simulink model "model"  (R2014a)
(part 5 of 6)

  bus544 : powerlib/Measurements/Load Flow Bus  LConnTagsString=a  ID=bus544  Vbase=132000  Vref=1  Vangle=0  VLF=1  angleLF=0
      settings: AttributesFormatString=|
      | %<ID>
      | %<Vbase>V
      | %<VLF>pu
      | %<angleLF>deg.
      | %<Name>
  bus545 : powerlib/Measurements/Load Flow Bus  LConnTagsString=a  ID=bus545  Vbase=132000  Vref=1  Vangle=0  VLF=1  angleLF=0
      settings: AttributesFormatString=|
      | %<ID>
      | %<Vbase>V
      | %<VLF>pu
      | %<angleLF>deg.
      | %<Name>
  bus546 : powerlib/Measurements/Load Flow Bus  LConnTagsString=a  ID=bus546  Vbase=132000  Vref=1  Vangle=0  VLF=1  angleLF=0
      settings: AttributesFormatString=|
      | %<ID>
      | %<Vbase>V
      | %<VLF>pu
      | %<angleLF>deg.
      | %<Name>
  bus547 : powerlib/Measurements/Load Flow Bus  LConnTagsString=a  ID=bus547  Vbase=132000  Vref=1  Vangle=0  VLF=1  angleLF=0
      settings: AttributesFormatString=|
      | %<ID>
      | %<Vbase>V
      | %<VLF>pu
      | %<angleLF>deg.
      | %<Name>
  bus548 : powerlib/Measurements/Load Flow Bus  LConnTagsString=a  ID=bus548  Vbase=132000  Vref=1  Vangle=0  VLF=1  angleLF=0
      settings: AttributesFormatString=|
      | %<ID>
      | %<Vbase>V
      | %<VLF>pu
      | %<angleLF>deg.
      | %<Name>
  bus549 : powerlib/Measurements/Load Flow Bus  LConnTagsString=a  ID=bus549  Vbase=132000  Vref=1  Vangle=0  VLF=1  angleLF=0
      settings: AttributesFormatString=|
      | %<ID>
      | %<Vbase>V
      | %<VLF>pu
      | %<angleLF>deg.
      | %<Name>
  bus55 : powerlib/Measurements/Load Flow Bus  LConnTagsString=a  ID=bus55  Vbase=132000  Vref=1  Vangle=0  VLF=1  angleLF=0
      settings: AttributesFormatString=|
      | %<ID>
      | %<Vbase>V
      | %<VLF>pu
      | %<angleLF>deg.
      | %<Name>
  bus550 : powerlib/Measurements/Load Flow Bus  LConnTagsString=a  ID=bus550  Vbase=132000  Vref=1  Vangle=0  VLF=1  angleLF=0
      settings: AttributesFormatString=|
      | %<ID>
      | %<Vbase>V
      | %<VLF>pu
      | %<angleLF>deg.
      | %<Name>
  bus551 : powerlib/Measurements/Load Flow Bus  LConnTagsString=a  ID=bus551  Vbase=132000  Vref=1  Vangle=0  VLF=1  angleLF=0
      settings: AttributesFormatString=|
      | %<ID>
      | %<Vbase>V
      | %<VLF>pu
      | %<angleLF>deg.
      | %<Name>
  bus552 : powerlib/Measurements/Load Flow Bus  LConnTagsString=a  ID=bus552  Vbase=132000  Vref=1  Vangle=0  VLF=1  angleLF=0
      settings: AttributesFormatString=|
      | %<ID>
      | %<Vbase>V
      | %<VLF>pu
      | %<angleLF>deg.
      | %<Name>
  bus553 : powerlib/Measurements/Load Flow Bus  LConnTagsString=a  ID=bus553  Vbase=132000  Vref=1  Vangle=0  VLF=1  angleLF=0
      settings: AttributesFormatString=|
      | %<ID>
      | %<Vbase>V
      | %<VLF>pu
      | %<angleLF>deg.
      | %<Name>
  bus554 : powerlib/Measurements/Load Flow Bus  LConnTagsString=a  ID=bus554  Vbase=132000  Vref=1  Vangle=0  VLF=1  angleLF=0
      settings: AttributesFormatString=|
      | %<ID>
      | %<Vbase>V
      | %<VLF>pu
      | %<angleLF>deg.
      | %<Name>
  bus555 : powerlib/Measurements/Load Flow Bus  LConnTagsString=a  ID=bus555  Vbase=132000  Vref=1  Vangle=0  VLF=1  angleLF=0
      settings: AttributesFormatString=|
      | %<ID>
      | %<Vbase>V
      | %<VLF>pu
      | %<angleLF>deg.
      | %<Name>
  bus556 : powerlib/Measurements/Load Flow Bus  LConnTagsString=a  ID=bus556  Vbase=220000  Vref=1  Vangle=0  VLF=1  angleLF=0
      settings: AttributesFormatString=|
      | %<ID>
      | %<Vbase>V
      | %<VLF>pu
      | %<angleLF>deg.
      | %<Name>
  bus557 : powerlib/Measurements/Load Flow Bus  LConnTagsString=a  ID=bus557  Vbase=220000  Vref=1  Vangle=0  VLF=1  angleLF=0
      settings: AttributesFormatString=|
      | %<ID>
      | %<Vbase>V
      | %<VLF>pu
      | %<angleLF>deg.
      | %<Name>
  bus558 : powerlib/Measurements/Load Flow Bus  LConnTagsString=a  ID=bus558  Vbase=220000  Vref=1  Vangle=0  VLF=1  angleLF=0
      settings: AttributesFormatString=|
      | %<ID>
      | %<Vbase>V
      | %<VLF>pu
      | %<angleLF>deg.
      | %<Name>
  bus559 : powerlib/Measurements/Load Flow Bus  LConnTagsString=a  ID=bus559  Vbase=220000  Vref=1  Vangle=0  VLF=1  angleLF=0
      settings: AttributesFormatString=|
      | %<ID>
      | %<Vbase>V
      | %<VLF>pu
      | %<angleLF>deg.
      | %<Name>
  bus56 : powerlib/Measurements/Load Flow Bus  LConnTagsString=a  ID=bus56  Vbase=132000  Vref=1  Vangle=0  VLF=1  angleLF=0
      settings: AttributesFormatString=|
      | %<ID>
      | %<Vbase>V
      | %<VLF>pu
      | %<angleLF>deg.
      | %<Name>
  bus560 : powerlib/Measurements/Load Flow Bus  LConnTagsString=a  ID=bus560  Vbase=220000  Vref=1  Vangle=0  VLF=1  angleLF=0
      settings: AttributesFormatString=|
      | %<ID>
      | %<Vbase>V
      | %<VLF>pu
      | %<angleLF>deg.
      | %<Name>
  bus561 : powerlib/Measurements/Load Flow Bus  LConnTagsString=a  ID=bus561  Vbase=220000  Vref=1  Vangle=0  VLF=1  angleLF=0
      settings: AttributesFormatString=|
      | %<ID>
      | %<Vbase>V
      | %<VLF>pu
      | %<angleLF>deg.
      | %<Name>
  bus562 : powerlib/Measurements/Load Flow Bus  LConnTagsString=a  ID=bus562  Vbase=220000  Vref=1  Vangle=0  VLF=1  angleLF=0
      settings: AttributesFormatString=|
      | %<ID>
      | %<Vbase>V
      | %<VLF>pu
      | %<angleLF>deg.
      | %<Name>
  bus563 : powerlib/Measurements/Load Flow Bus  LConnTagsString=a  ID=bus563  Vbase=220000  Vref=1  Vangle=0  VLF=1  angleLF=0
      settings: AttributesFormatString=|
      | %<ID>
      | %<Vbase>V
      | %<VLF>pu
      | %<angleLF>deg.
      | %<Name>
  bus564 : powerlib/Measurements/Load Flow Bus  LConnTagsString=a  ID=bus564  Vbase=220000  Vref=1  Vangle=0  VLF=1  angleLF=0
      settings: AttributesFormatString=|
      | %<ID>
      | %<Vbase>V
      | %<VLF>pu
      | %<angleLF>deg.
      | %<Name>
  bus565 : powerlib/Measurements/Load Flow Bus  LConnTagsString=a  ID=bus565  Vbase=220000  Vref=1  Vangle=0  VLF=1  angleLF=0
      settings: AttributesFormatString=|
      | %<ID>
      | %<Vbase>V
      | %<VLF>pu
      | %<angleLF>deg.
      | %<Name>
  bus566 : powerlib/Measurements/Load Flow Bus  LConnTagsString=a  ID=bus566  Vbase=220000  Vref=1  Vangle=0  VLF=1  angleLF=0
      settings: AttributesFormatString=|
      | %<ID>
      | %<Vbase>V
      | %<VLF>pu
      | %<angleLF>deg.
      | %<Name>
  bus567 : powerlib/Measurements/Load Flow Bus  LConnTagsString=a  ID=bus567  Vbase=220000  Vref=1  Vangle=0  VLF=1  angleLF=0
      settings: AttributesFormatString=|
      | %<ID>
      | %<Vbase>V
      | %<VLF>pu
      | %<angleLF>deg.
      | %<Name>
  bus568 : powerlib/Measurements/Load Flow Bus  LConnTagsString=a  ID=bus568  Vbase=220000  Vref=1  Vangle=0  VLF=1  angleLF=0
      settings: AttributesFormatString=|
      | %<ID>
      | %<Vbase>V
      | %<VLF>pu
      | %<angleLF>deg.
      | %<Name>
  bus569 : powerlib/Measurements/Load Flow Bus  LConnTagsString=a  ID=bus569  Vbase=220000  Vref=1  Vangle=0  VLF=1  angleLF=0
      settings: AttributesFormatString=|
      | %<ID>
      | %<Vbase>V
      | %<VLF>pu
      | %<angleLF>deg.
      | %<Name>
  bus57 : powerlib/Measurements/Load Flow Bus  LConnTagsString=a  ID=bus57  Vbase=132000  Vref=1  Vangle=0  VLF=1  angleLF=0
      settings: AttributesFormatString=|
      | %<ID>
      | %<Vbase>V
      | %<VLF>pu
      | %<angleLF>deg.
      | %<Name>
  bus570 : powerlib/Measurements/Load Flow Bus  LConnTagsString=a  ID=bus570  Vbase=220000  Vref=1  Vangle=0  VLF=1  angleLF=0
      settings: AttributesFormatString=|
      | %<ID>
      | %<Vbase>V
      | %<VLF>pu
      | %<angleLF>deg.
      | %<Name>
  bus571 : powerlib/Measurements/Load Flow Bus  LConnTagsString=a  ID=bus571  Vbase=220000  Vref=1  Vangle=0  VLF=1  angleLF=0
      settings: AttributesFormatString=|
      | %<ID>
      | %<Vbase>V
      | %<VLF>pu
      | %<angleLF>deg.
      | %<Name>
  bus572 : powerlib/Measurements/Load Flow Bus  LConnTagsString=a  ID=bus572  Vbase=220000  Vref=1  Vangle=0  VLF=1  angleLF=0
      settings: AttributesFormatString=|
      | %<ID>
      | %<Vbase>V
      | %<VLF>pu
      | %<angleLF>deg.
      | %<Name>
  bus573 : powerlib/Measurements/Load Flow Bus  LConnTagsString=a  ID=bus573  Vbase=220000  Vref=1  Vangle=0  VLF=1  angleLF=0
      settings: AttributesFormatString=|
      | %<ID>
      | %<Vbase>V
      | %<VLF>pu
      | %<angleLF>deg.
      | %<Name>
  bus574 : powerlib/Measurements/Load Flow Bus  LConnTagsString=a  ID=bus574  Vbase=220000  Vref=1  Vangle=0  VLF=1  angleLF=0
      settings: AttributesFormatString=|
      | %<ID>
      | %<Vbase>V
      | %<VLF>pu
      | %<angleLF>deg.
      | %<Name>
  bus575 : powerlib/Measurements/Load Flow Bus  LConnTagsString=a  ID=bus575  Vbase=220000  Vref=1  Vangle=0  VLF=1  angleLF=0
      settings: AttributesFormatString=|
      | %<ID>
      | %<Vbase>V
      | %<VLF>pu
      | %<angleLF>deg.
      | %<Name>
  bus576 : powerlib/Measurements/Load Flow Bus  LConnTagsString=a  ID=bus576  Vbase=220000  Vref=1  Vangle=0  VLF=1  angleLF=0
      settings: AttributesFormatString=|
      | %<ID>
      | %<Vbase>V
      | %<VLF>pu
      | %<angleLF>deg.
      | %<Name>
  bus577 : powerlib/Measurements/Load Flow Bus  LConnTagsString=a  ID=bus577  Vbase=220000  Vref=1  Vangle=0  VLF=1  angleLF=0
      settings: AttributesFormatString=|
      | %<ID>
      | %<Vbase>V
      | %<VLF>pu
      | %<angleLF>deg.
      | %<Name>
  bus578 : powerlib/Measurements/Load Flow Bus  LConnTagsString=a  ID=bus578  Vbase=220000  Vref=1  Vangle=0  VLF=1  angleLF=0
      settings: AttributesFormatString=|
      | %<ID>
      | %<Vbase>V
      | %<VLF>pu
      | %<angleLF>deg.
      | %<Name>
  bus579 : powerlib/Measurements/Load Flow Bus  LConnTagsString=a  ID=bus579  Vbase=220000  Vref=1  Vangle=0  VLF=1  angleLF=0
      settings: AttributesFormatString=|
      | %<ID>
      | %<Vbase>V
      | %<VLF>pu
      | %<angleLF>deg.
      | %<Name>
  bus58 : powerlib/Measurements/Load Flow Bus  LConnTagsString=a  ID=bus58  Vbase=132000  Vref=1  Vangle=0  VLF=1  angleLF=0
      settings: AttributesFormatString=|
      | %<ID>
      | %<Vbase>V
      | %<VLF>pu
      | %<angleLF>deg.
      | %<Name>
  bus580 : powerlib/Measurements/Load Flow Bus  LConnTagsString=a  ID=bus580  Vbase=220000  Vref=1  Vangle=0  VLF=1  angleLF=0
      settings: AttributesFormatString=|
      | %<ID>
      | %<Vbase>V
      | %<VLF>pu
      | %<angleLF>deg.
      | %<Name>
  bus581 : powerlib/Measurements/Load Flow Bus  LConnTagsString=a  ID=bus581  Vbase=220000  Vref=1  Vangle=0  VLF=1  angleLF=0
      settings: AttributesFormatString=|
      | %<ID>
      | %<Vbase>V
      | %<VLF>pu
      | %<angleLF>deg.
      | %<Name>
  bus582 : powerlib/Measurements/Load Flow Bus  LConnTagsString=a  ID=bus582  Vbase=220000  Vref=1  Vangle=0  VLF=1  angleLF=0
      settings: AttributesFormatString=|
      | %<ID>
      | %<Vbase>V
      | %<VLF>pu
      | %<angleLF>deg.
      | %<Name>
  bus583 : powerlib/Measurements/Load Flow Bus  LConnTagsString=a  ID=bus583  Vbase=220000  Vref=1  Vangle=0  VLF=1  angleLF=0
      settings: AttributesFormatString=|
      | %<ID>
      | %<Vbase>V
      | %<VLF>pu
      | %<angleLF>deg.
      | %<Name>
  bus584 : powerlib/Measurements/Load Flow Bus  LConnTagsString=a  ID=bus584  Vbase=220000  Vref=1  Vangle=0  VLF=1  angleLF=0
      settings: AttributesFormatString=|
      | %<ID>
      | %<Vbase>V
      | %<VLF>pu
      | %<angleLF>deg.
      | %<Name>
  bus585 : powerlib/Measurements/Load Flow Bus  LConnTagsString=a  ID=bus585  Vbase=220000  Vref=1  Vangle=0  VLF=1  angleLF=0
      settings: AttributesFormatString=|
      | %<ID>
      | %<Vbase>V
      | %<VLF>pu
      | %<angleLF>deg.
      | %<Name>
  bus586 : powerlib/Measurements/Load Flow Bus  LConnTagsString=a  ID=bus586  Vbase=230000  Vref=1  Vangle=0  VLF=1  angleLF=0
      settings: AttributesFormatString=|
      | %<ID>
      | %<Vbase>V
      | %<VLF>pu
      | %<angleLF>deg.
      | %<Name>
  bus587 : powerlib/Measurements/Load Flow Bus  LConnTagsString=a  ID=bus587  Vbase=230000  Vref=1  Vangle=0  VLF=1  angleLF=0
      settings: AttributesFormatString=|
      | %<ID>
      | %<Vbase>V
      | %<VLF>pu
      | %<angleLF>deg.
      | %<Name>
  bus588 : powerlib/Measurements/Load Flow Bus  LConnTagsString=a  ID=bus588  Vbase=230000  Vref=1  Vangle=0  VLF=1  angleLF=0
      settings: AttributesFormatString=|
      | %<ID>
      | %<Vbase>V
      | %<VLF>pu
      | %<angleLF>deg.
      | %<Name>
  bus589 : powerlib/Measurements/Load Flow Bus  LConnTagsString=a  ID=bus589  Vbase=230000  Vref=1  Vangle=0  VLF=1  angleLF=0
      settings: AttributesFormatString=|
      | %<ID>
      | %<Vbase>V
      | %<VLF>pu
      | %<angleLF>deg.
      | %<Name>
  bus59 : powerlib/Measurements/Load Flow Bus  LConnTagsString=a  ID=bus59  Vbase=132000  Vref=1  Vangle=0  VLF=1  angleLF=0
      settings: AttributesFormatString=|
      | %<ID>
      | %<Vbase>V
      | %<VLF>pu
      | %<angleLF>deg.
      | %<Name>
  bus590 : powerlib/Measurements/Load Flow Bus  LConnTagsString=a  ID=bus590  Vbase=230000  Vref=1  Vangle=0  VLF=1  angleLF=0
      settings: AttributesFormatString=|
      | %<ID>
      | %<Vbase>V
      | %<VLF>pu
      | %<angleLF>deg.
      | %<Name>
  bus591 : powerlib/Measurements/Load Flow Bus  LConnTagsString=a  ID=bus591  Vbase=230000  Vref=1  Vangle=0  VLF=1  angleLF=0
      settings: AttributesFormatString=|
      | %<ID>
      | %<Vbase>V
      | %<VLF>pu
      | %<angleLF>deg.
      | %<Name>
  bus592 : powerlib/Measurements/Load Flow Bus  LConnTagsString=a  ID=bus592  Vbase=230000  Vref=1  Vangle=0  VLF=1  angleLF=0
      settings: AttributesFormatString=|
      | %<ID>
      | %<Vbase>V
      | %<VLF>pu
      | %<angleLF>deg.
      | %<Name>
  bus593 : powerlib/Measurements/Load Flow Bus  LConnTagsString=a  ID=bus593  Vbase=230000  Vref=1  Vangle=0  VLF=1  angleLF=0
      settings: AttributesFormatString=|
      | %<ID>
      | %<Vbase>V
      | %<VLF>pu
      | %<angleLF>deg.
      | %<Name>
  bus594 : powerlib/Measurements/Load Flow Bus  LConnTagsString=a  ID=bus594  Vbase=230000  Vref=1  Vangle=0  VLF=1  angleLF=0
      settings: AttributesFormatString=|
      | %<ID>
      | %<Vbase>V
      | %<VLF>pu
      | %<angleLF>deg.
      | %<Name>
  bus595 : powerlib/Measurements/Load Flow Bus  LConnTagsString=a  ID=bus595  Vbase=230000  Vref=1  Vangle=0  VLF=1  angleLF=0
      settings: AttributesFormatString=|
      | %<ID>
      | %<Vbase>V
      | %<VLF>pu
      | %<angleLF>deg.
      | %<Name>
  bus596 : powerlib/Measurements/Load Flow Bus  LConnTagsString=a  ID=bus596  Vbase=230000  Vref=1  Vangle=0  VLF=1  angleLF=0
      settings: AttributesFormatString=|
      | %<ID>
      | %<Vbase>V
      | %<VLF>pu
      | %<angleLF>deg.
      | %<Name>
  bus597 : powerlib/Measurements/Load Flow Bus  LConnTagsString=a  ID=bus597  Vbase=230000  Vref=1  Vangle=0  VLF=1  angleLF=0
      settings: AttributesFormatString=|
      | %<ID>
      | %<Vbase>V
      | %<VLF>pu
      | %<angleLF>deg.
      | %<Name>
  bus598 : powerlib/Measurements/Load Flow Bus  LConnTagsString=a  ID=bus598  Vbase=230000  Vref=1  Vangle=0  VLF=1  angleLF=0
      settings: AttributesFormatString=|
      | %<ID>
      | %<Vbase>V
      | %<VLF>pu
      | %<angleLF>deg.
      | %<Name>
  bus599 : powerlib/Measurements/Load Flow Bus  LConnTagsString=a  ID=bus599  Vbase=230000  Vref=1  Vangle=0  VLF=1  angleLF=0
      settings: AttributesFormatString=|
      | %<ID>
      | %<Vbase>V
      | %<VLF>pu
      | %<angleLF>deg.
      | %<Name>
  bus6 : powerlib/Measurements/Load Flow Bus  LConnTagsString=a  ID=bus6  Vbase=132000  Vref=1  Vangle=0  VLF=1  angleLF=0
      settings: AttributesFormatString=|
      | %<ID>
      | %<Vbase>V
      | %<VLF>pu
      | %<angleLF>deg.
      | %<Name>
  bus60 : powerlib/Measurements/Load Flow Bus  LConnTagsString=a  ID=bus60  Vbase=132000  Vref=1  Vangle=0  VLF=1  angleLF=0
      settings: AttributesFormatString=|
      | %<ID>
      | %<Vbase>V
      | %<VLF>pu
      | %<angleLF>deg.
      | %<Name>
  bus600 : powerlib/Measurements/Load Flow Bus  LConnTagsString=a  ID=bus600  Vbase=230000  Vref=1  Vangle=0  VLF=1  angleLF=0
      settings: AttributesFormatString=|
      | %<ID>
      | %<Vbase>V
      | %<VLF>pu
      | %<angleLF>deg.
      | %<Name>
  bus601 : powerlib/Measurements/Load Flow Bus  LConnTagsString=a  ID=bus601  Vbase=230000  Vref=1  Vangle=0  VLF=1  angleLF=0
      settings: AttributesFormatString=|
      | %<ID>
      | %<Vbase>V
      | %<VLF>pu
      | %<angleLF>deg.
      | %<Name>
  bus602 : powerlib/Measurements/Load Flow Bus  LConnTagsString=a  ID=bus602  Vbase=230000  Vref=1  Vangle=0  VLF=1  angleLF=0
      settings: AttributesFormatString=|
      | %<ID>
      | %<Vbase>V
      | %<VLF>pu
      | %<angleLF>deg.
      | %<Name>
  bus603 : powerlib/Measurements/Load Flow Bus  LConnTagsString=a  ID=bus603  Vbase=230000  Vref=1  Vangle=0  VLF=1  angleLF=0
      settings: AttributesFormatString=|
      | %<ID>
      | %<Vbase>V
      | %<VLF>pu
      | %<angleLF>deg.
      | %<Name>
  bus604 : powerlib/Measurements/Load Flow Bus  LConnTagsString=a  ID=bus604  Vbase=230000  Vref=1  Vangle=0  VLF=1  angleLF=0
      settings: AttributesFormatString=|
      | %<ID>
      | %<Vbase>V
      | %<VLF>pu
      | %<angleLF>deg.
      | %<Name>
  bus605 : powerlib/Measurements/Load Flow Bus  LConnTagsString=a  ID=bus605  Vbase=230000  Vref=1  Vangle=0  VLF=1  angleLF=0
      settings: AttributesFormatString=|
      | %<ID>
      | %<Vbase>V
      | %<VLF>pu
      | %<angleLF>deg.
      | %<Name>
  bus606 : powerlib/Measurements/Load Flow Bus  LConnTagsString=a  ID=bus606  Vbase=230000  Vref=1  Vangle=0  VLF=1  angleLF=0
      settings: AttributesFormatString=|
      | %<ID>
      | %<Vbase>V
      | %<VLF>pu
      | %<angleLF>deg.
      | %<Name>
  bus607 : powerlib/Measurements/Load Flow Bus  LConnTagsString=a  ID=bus607  Vbase=275000  Vref=1  Vangle=0  VLF=1  angleLF=0
      settings: AttributesFormatString=|
      | %<ID>
      | %<Vbase>V
      | %<VLF>pu
      | %<angleLF>deg.
      | %<Name>
  bus608 : powerlib/Measurements/Load Flow Bus  LConnTagsString=a  ID=bus608  Vbase=275000  Vref=1  Vangle=0  VLF=1  angleLF=0
      settings: AttributesFormatString=|
      | %<ID>
      | %<Vbase>V
      | %<VLF>pu
      | %<angleLF>deg.
      | %<Name>
  bus609 : powerlib/Measurements/Load Flow Bus  LConnTagsString=a  ID=bus609  Vbase=275000  Vref=1  Vangle=0  VLF=1  angleLF=0
      settings: AttributesFormatString=|
      | %<ID>
      | %<Vbase>V
      | %<VLF>pu
      | %<angleLF>deg.
      | %<Name>
  bus61 : powerlib/Measurements/Load Flow Bus  LConnTagsString=a  ID=bus61  Vbase=132000  Vref=1  Vangle=0  VLF=1  angleLF=0
      settings: AttributesFormatString=|
      | %<ID>
      | %<Vbase>V
      | %<VLF>pu
      | %<angleLF>deg.
      | %<Name>
  bus610 : powerlib/Measurements/Load Flow Bus  LConnTagsString=a  ID=bus610  Vbase=275000  Vref=1  Vangle=0  VLF=1  angleLF=0
      settings: AttributesFormatString=|
      | %<ID>
      | %<Vbase>V
      | %<VLF>pu
      | %<angleLF>deg.
      | %<Name>
  bus611 : powerlib/Measurements/Load Flow Bus  LConnTagsString=a  ID=bus611  Vbase=275000  Vref=1  Vangle=0  VLF=1  angleLF=0
      settings: AttributesFormatString=|
      | %<ID>
      | %<Vbase>V
      | %<VLF>pu
      | %<angleLF>deg.
      | %<Name>
  bus612 : powerlib/Measurements/Load Flow Bus  LConnTagsString=a  ID=bus612  Vbase=275000  Vref=1  Vangle=0  VLF=1  angleLF=0
      settings: AttributesFormatString=|
      | %<ID>
      | %<Vbase>V
      | %<VLF>pu
      | %<angleLF>deg.
      | %<Name>
  bus613 : powerlib/Measurements/Load Flow Bus  LConnTagsString=a  ID=bus613  Vbase=275000  Vref=1  Vangle=0  VLF=1  angleLF=0
      settings: AttributesFormatString=|
      | %<ID>
      | %<Vbase>V
      | %<VLF>pu
      | %<angleLF>deg.
      | %<Name>
  bus614 : powerlib/Measurements/Load Flow Bus  LConnTagsString=a  ID=bus614  Vbase=275000  Vref=1  Vangle=0  VLF=1  angleLF=0
      settings: AttributesFormatString=|
      | %<ID>
      | %<Vbase>V
      | %<VLF>pu
      | %<angleLF>deg.
      | %<Name>
  bus615 : powerlib/Measurements/Load Flow Bus  LConnTagsString=a  ID=bus615  Vbase=275000  Vref=1  Vangle=0  VLF=1  angleLF=0
      settings: AttributesFormatString=|
      | %<ID>
      | %<Vbase>V
      | %<VLF>pu
      | %<angleLF>deg.
      | %<Name>
  bus616 : powerlib/Measurements/Load Flow Bus  LConnTagsString=a  ID=bus616  Vbase=275000  Vref=1  Vangle=0  VLF=1  angleLF=0
      settings: AttributesFormatString=|
      | %<ID>
      | %<Vbase>V
      | %<VLF>pu
      | %<angleLF>deg.
      | %<Name>
  bus617 : powerlib/Measurements/Load Flow Bus  LConnTagsString=a  ID=bus617  Vbase=275000  Vref=1  Vangle=0  VLF=1  angleLF=0
      settings: AttributesFormatString=|
      | %<ID>
      | %<Vbase>V
      | %<VLF>pu
      | %<angleLF>deg.
      | %<Name>
  bus618 : powerlib/Measurements/Load Flow Bus  LConnTagsString=a  ID=bus618  Vbase=275000  Vref=1  Vangle=0  VLF=1  angleLF=0
      settings: AttributesFormatString=|
      | %<ID>
      | %<Vbase>V
      | %<VLF>pu
      | %<angleLF>deg.
      | %<Name>
  bus619 : powerlib/Measurements/Load Flow Bus  LConnTagsString=a  ID=bus619  Vbase=380000  Vref=1  Vangle=0  VLF=1  angleLF=0
      settings: AttributesFormatString=|
      | %<ID>
      | %<Vbase>V
      | %<VLF>pu
      | %<angleLF>deg.
      | %<Name>
  bus62 : powerlib/Measurements/Load Flow Bus  LConnTagsString=a  ID=bus62  Vbase=132000  Vref=1  Vangle=0  VLF=1  angleLF=0
      settings: AttributesFormatString=|
      | %<ID>
      | %<Vbase>V
      | %<VLF>pu
      | %<angleLF>deg.
      | %<Name>
  bus620 : powerlib/Measurements/Load Flow Bus  LConnTagsString=a  ID=bus620  Vbase=380000  Vref=1  Vangle=0  VLF=1  angleLF=0
      settings: AttributesFormatString=|
      | %<ID>
      | %<Vbase>V
      | %<VLF>pu
      | %<angleLF>deg.
      | %<Name>
  bus621 : powerlib/Measurements/Load Flow Bus  LConnTagsString=a  ID=bus621  Vbase=380000  Vref=1  Vangle=0  VLF=1  angleLF=0
      settings: AttributesFormatString=|
      | %<ID>
      | %<Vbase>V
      | %<VLF>pu
      | %<angleLF>deg.
      | %<Name>
  bus622 : powerlib/Measurements/Load Flow Bus  LConnTagsString=a  ID=bus622  Vbase=380000  Vref=1  Vangle=0  VLF=1  angleLF=0
      settings: AttributesFormatString=|
      | %<ID>
      | %<Vbase>V
      | %<VLF>pu
      | %<angleLF>deg.
      | %<Name>
  bus623 : powerlib/Measurements/Load Flow Bus  LConnTagsString=a  ID=bus623  Vbase=380000  Vref=1  Vangle=0  VLF=1  angleLF=0
      settings: AttributesFormatString=|
      | %<ID>
      | %<Vbase>V
      | %<VLF>pu
      | %<angleLF>deg.
      | %<Name>
  bus624 : powerlib/Measurements/Load Flow Bus  LConnTagsString=a  ID=bus624  Vbase=380000  Vref=1  Vangle=0  VLF=1  angleLF=0
      settings: AttributesFormatString=|
      | %<ID>
      | %<Vbase>V
      | %<VLF>pu
      | %<angleLF>deg.
      | %<Name>
  bus625 : powerlib/Measurements/Load Flow Bus  LConnTagsString=a  ID=bus625  Vbase=380000  Vref=1  Vangle=0  VLF=1  angleLF=0
      settings: AttributesFormatString=|
      | %<ID>
      | %<Vbase>V
      | %<VLF>pu
      | %<angleLF>deg.
      | %<Name>
  bus626 : powerlib/Measurements/Load Flow Bus  LConnTagsString=a  ID=bus626  Vbase=380000  Vref=1  Vangle=0  VLF=1  angleLF=0
      settings: AttributesFormatString=|
      | %<ID>
      | %<Vbase>V
      | %<VLF>pu
      | %<angleLF>deg.
      | %<Name>
  bus627 : powerlib/Measurements/Load Flow Bus  LConnTagsString=a  ID=bus627  Vbase=380000  Vref=1  Vangle=0  VLF=1  angleLF=0
      settings: AttributesFormatString=|
      | %<ID>
      | %<Vbase>V
      | %<VLF>pu
      | %<angleLF>deg.
      | %<Name>
  bus628 : powerlib/Measurements/Load Flow Bus  LConnTagsString=a  ID=bus628  Vbase=380000  Vref=1  Vangle=0  VLF=1  angleLF=0
      settings: AttributesFormatString=|
      | %<ID>
      | %<Vbase>V
      | %<VLF>pu
      | %<angleLF>deg.
      | %<Name>
  bus629 : powerlib/Measurements/Load Flow Bus  LConnTagsString=a  ID=bus629  Vbase=380000  Vref=1  Vangle=0  VLF=1  angleLF=0
      settings: AttributesFormatString=|
      | %<ID>
      | %<Vbase>V
      | %<VLF>pu
      | %<angleLF>deg.
      | %<Name>
  bus63 : powerlib/Measurements/Load Flow Bus  LConnTagsString=a  ID=bus63  Vbase=132000  Vref=1  Vangle=0  VLF=1  angleLF=0
      settings: AttributesFormatString=|
      | %<ID>
      | %<Vbase>V
      | %<VLF>pu
      | %<angleLF>deg.
      | %<Name>
  bus630 : powerlib/Measurements/Load Flow Bus  LConnTagsString=a  ID=bus630  Vbase=380000  Vref=1  Vangle=0  VLF=1  angleLF=0
      settings: AttributesFormatString=|
      | %<ID>
      | %<Vbase>V
      | %<VLF>pu
      | %<angleLF>deg.
      | %<Name>
  bus631 : powerlib/Measurements/Load Flow Bus  LConnTagsString=a  ID=bus631  Vbase=380000  Vref=1  Vangle=0  VLF=1  angleLF=0
      settings: AttributesFormatString=|
      | %<ID>
      | %<Vbase>V
      | %<VLF>pu
      | %<angleLF>deg.
      | %<Name>
  bus632 : powerlib/Measurements/Load Flow Bus  LConnTagsString=a  ID=bus632  Vbase=380000  Vref=1  Vangle=0  VLF=1  angleLF=0
      settings: AttributesFormatString=|
      | %<ID>
      | %<Vbase>V
      | %<VLF>pu
      | %<angleLF>deg.
      | %<Name>
  bus633 : powerlib/Measurements/Load Flow Bus  LConnTagsString=a  ID=bus633  Vbase=380000  Vref=1  Vangle=0  VLF=1  angleLF=0
      settings: AttributesFormatString=|
      | %<ID>
      | %<Vbase>V
      | %<VLF>pu
      | %<angleLF>deg.
      | %<Name>
  bus634 : powerlib/Measurements/Load Flow Bus  LConnTagsString=a  ID=bus634  Vbase=380000  Vref=1  Vangle=0  VLF=1  angleLF=0
      settings: AttributesFormatString=|
      | %<ID>
      | %<Vbase>V
      | %<VLF>pu
      | %<angleLF>deg.
      | %<Name>
  bus635 : powerlib/Measurements/Load Flow Bus  LConnTagsString=a  ID=bus635  Vbase=380000  Vref=1  Vangle=0  VLF=1  angleLF=0
      settings: AttributesFormatString=|
      | %<ID>
      | %<Vbase>V
      | %<VLF>pu
      | %<angleLF>deg.
      | %<Name>
  bus636 : powerlib/Measurements/Load Flow Bus  LConnTagsString=a  ID=bus636  Vbase=380000  Vref=1  Vangle=0  VLF=1  angleLF=0
      settings: AttributesFormatString=|
      | %<ID>
      | %<Vbase>V
      | %<VLF>pu
      | %<angleLF>deg.
      | %<Name>
  bus637 : powerlib/Measurements/Load Flow Bus  LConnTagsString=a  ID=bus637  Vbase=380000  Vref=1  Vangle=0  VLF=1  angleLF=0
      settings: AttributesFormatString=|
      | %<ID>
      | %<Vbase>V
      | %<VLF>pu
      | %<angleLF>deg.
      | %<Name>
  bus638 : powerlib/Measurements/Load Flow Bus  LConnTagsString=a  ID=bus638  Vbase=380000  Vref=1  Vangle=0  VLF=1  angleLF=0
      settings: AttributesFormatString=|
      | %<ID>
      | %<Vbase>V
      | %<VLF>pu
      | %<angleLF>deg.
      | %<Name>
  bus639 : powerlib/Measurements/Load Flow Bus  LConnTagsString=a  ID=bus639  Vbase=380000  Vref=1  Vangle=0  VLF=1  angleLF=0
      settings: AttributesFormatString=|
      | %<ID>
      | %<Vbase>V
      | %<VLF>pu
      | %<angleLF>deg.
      | %<Name>
  bus64 : powerlib/Measurements/Load Flow Bus  LConnTagsString=a  ID=bus64  Vbase=132000  Vref=1  Vangle=0  VLF=1  angleLF=0
      settings: AttributesFormatString=|
      | %<ID>
      | %<Vbase>V
      | %<VLF>pu
      | %<angleLF>deg.
      | %<Name>
  bus640 : powerlib/Measurements/Load Flow Bus  LConnTagsString=a  ID=bus640  Vbase=380000  Vref=1  Vangle=0  VLF=1  angleLF=0
      settings: AttributesFormatString=|
      | %<ID>
      | %<Vbase>V
      | %<VLF>pu
      | %<angleLF>deg.
      | %<Name>
  bus641 : powerlib/Measurements/Load Flow Bus  LConnTagsString=a  ID=bus641  Vbase=380000  Vref=1  Vangle=0  VLF=1  angleLF=0
      settings: AttributesFormatString=|
      | %<ID>
      | %<Vbase>V
      | %<VLF>pu
      | %<angleLF>deg.
      | %<Name>
  bus642 : powerlib/Measurements/Load Flow Bus  LConnTagsString=a  ID=bus642  Vbase=380000  Vref=1  Vangle=0  VLF=1  angleLF=0
      settings: AttributesFormatString=|
      | %<ID>
      | %<Vbase>V
      | %<VLF>pu
      | %<angleLF>deg.
      | %<Name>
  bus643 : powerlib/Measurements/Load Flow Bus  LConnTagsString=a  ID=bus643  Vbase=380000  Vref=1  Vangle=0  VLF=1  angleLF=0
      settings: AttributesFormatString=|
      | %<ID>
      | %<Vbase>V
      | %<VLF>pu
      | %<angleLF>deg.
      | %<Name>
  bus644 : powerlib/Measurements/Load Flow Bus  LConnTagsString=a  ID=bus644  Vbase=380000  Vref=1  Vangle=0  VLF=1  angleLF=0
      settings: AttributesFormatString=|
      | %<ID>
      | %<Vbase>V
      | %<VLF>pu
      | %<angleLF>deg.
      | %<Name>
  bus645 : powerlib/Measurements/Load Flow Bus  LConnTagsString=a  ID=bus645  Vbase=380000  Vref=1  Vangle=0  VLF=1  angleLF=0
      settings: AttributesFormatString=|
      | %<ID>
      | %<Vbase>V
      | %<VLF>pu
      | %<angleLF>deg.
      | %<Name>
  bus646 : powerlib/Measurements/Load Flow Bus  LConnTagsString=a  ID=bus646  Vbase=380000  Vref=1  Vangle=0  VLF=1  angleLF=0
      settings: AttributesFormatString=|
      | %<ID>
      | %<Vbase>V
      | %<VLF>pu
      | %<angleLF>deg.
      | %<Name>
  bus647 : powerlib/Measurements/Load Flow Bus  LConnTagsString=a  ID=bus647  Vbase=380000  Vref=1  Vangle=0  VLF=1  angleLF=0
      settings: AttributesFormatString=|
      | %<ID>
      | %<Vbase>V
      | %<VLF>pu
      | %<angleLF>deg.
      | %<Name>
  bus648 : powerlib/Measurements/Load Flow Bus  LConnTagsString=a  ID=bus648  Vbase=380000  Vref=1  Vangle=0  VLF=1  angleLF=0
      settings: AttributesFormatString=|
      | %<ID>
      | %<Vbase>V
      | %<VLF>pu
      | %<angleLF>deg.
      | %<Name>
  bus649 : powerlib/Measurements/Load Flow Bus  LConnTagsString=a  ID=bus649  Vbase=380000  Vref=1  Vangle=0  VLF=1  angleLF=0
      settings: AttributesFormatString=|
      | %<ID>
      | %<Vbase>V
      | %<VLF>pu
      | %<angleLF>deg.
      | %<Name>
  bus65 : powerlib/Measurements/Load Flow Bus  LConnTagsString=a  ID=bus65  Vbase=132000  Vref=1  Vangle=0  VLF=1  angleLF=0
      settings: AttributesFormatString=|
      | %<ID>
      | %<Vbase>V
      | %<VLF>pu
      | %<angleLF>deg.
      | %<Name>
  bus650 : powerlib/Measurements/Load Flow Bus  LConnTagsString=a  ID=bus650  Vbase=380000  Vref=1  Vangle=0  VLF=1  angleLF=0
      settings: AttributesFormatString=|
      | %<ID>
      | %<Vbase>V
      | %<VLF>pu
      | %<angleLF>deg.
      | %<Name>
  bus651 : powerlib/Measurements/Load Flow Bus  LConnTagsString=a  ID=bus651  Vbase=380000  Vref=1  Vangle=0  VLF=1  angleLF=0
      settings: AttributesFormatString=|
      | %<ID>
      | %<Vbase>V
      | %<VLF>pu
      | %<angleLF>deg.
      | %<Name>
  bus652 : powerlib/Measurements/Load Flow Bus  LConnTagsString=a  ID=bus652  Vbase=380000  Vref=1  Vangle=0  VLF=1  angleLF=0
      settings: AttributesFormatString=|
      | %<ID>
      | %<Vbase>V
      | %<VLF>pu
      | %<angleLF>deg.
      | %<Name>
  bus653 : powerlib/Measurements/Load Flow Bus  LConnTagsString=a  ID=bus653  Vbase=400000  Vref=1  Vangle=0  VLF=1  angleLF=0
      settings: AttributesFormatString=|
      | %<ID>
      | %<Vbase>V
      | %<VLF>pu
      | %<angleLF>deg.
      | %<Name>
  bus654 : powerlib/Measurements/Load Flow Bus  LConnTagsString=a  ID=bus654  Vbase=400000  Vref=1  Vangle=0  VLF=1  angleLF=0
      settings: AttributesFormatString=|
      | %<ID>
      | %<Vbase>V
      | %<VLF>pu
      | %<angleLF>deg.
      | %<Name>
  bus655 : powerlib/Measurements/Load Flow Bus  LConnTagsString=a  ID=bus655  Vbase=400000  Vref=1  Vangle=0  VLF=1  angleLF=0
      settings: AttributesFormatString=|
      | %<ID>
      | %<Vbase>V
      | %<VLF>pu
      | %<angleLF>deg.
      | %<Name>
  bus656 : powerlib/Measurements/Load Flow Bus  LConnTagsString=a  ID=bus656  Vbase=400000  Vref=1  Vangle=0  VLF=1  angleLF=0
      settings: AttributesFormatString=|
      | %<ID>
      | %<Vbase>V
      | %<VLF>pu
      | %<angleLF>deg.
      | %<Name>
  bus657 : powerlib/Measurements/Load Flow Bus  LConnTagsString=a  ID=bus657  Vbase=400000  Vref=1  Vangle=0  VLF=1  angleLF=0
      settings: AttributesFormatString=|
      | %<ID>
      | %<Vbase>V
      | %<VLF>pu
      | %<angleLF>deg.
      | %<Name>
  bus658 : powerlib/Measurements/Load Flow Bus  LConnTagsString=a  ID=bus658  Vbase=400000  Vref=1  Vangle=0  VLF=1  angleLF=0
      settings: AttributesFormatString=|
      | %<ID>
      | %<Vbase>V
      | %<VLF>pu
      | %<angleLF>deg.
      | %<Name>
  bus659 : powerlib/Measurements/Load Flow Bus  LConnTagsString=a  ID=bus659  Vbase=400000  Vref=1  Vangle=0  VLF=1  angleLF=0
      settings: AttributesFormatString=|
      | %<ID>
      | %<Vbase>V
      | %<VLF>pu
      | %<angleLF>deg.
      | %<Name>
  bus66 : powerlib/Measurements/Load Flow Bus  LConnTagsString=a  ID=bus66  Vbase=132000  Vref=1  Vangle=0  VLF=1  angleLF=0
      settings: AttributesFormatString=|
      | %<ID>
      | %<Vbase>V
      | %<VLF>pu
      | %<angleLF>deg.
      | %<Name>
  bus660 : powerlib/Measurements/Load Flow Bus  LConnTagsString=a  ID=bus660  Vbase=400000  Vref=1  Vangle=0  VLF=1  angleLF=0
      settings: AttributesFormatString=|
      | %<ID>
      | %<Vbase>V
      | %<VLF>pu
      | %<angleLF>deg.
      | %<Name>
  bus661 : powerlib/Measurements/Load Flow Bus  LConnTagsString=a  ID=bus661  Vbase=400000  Vref=1  Vangle=0  VLF=1  angleLF=0
      settings: AttributesFormatString=|
      | %<ID>
      | %<Vbase>V
      | %<VLF>pu
      | %<angleLF>deg.
      | %<Name>
  bus662 : powerlib/Measurements/Load Flow Bus  LConnTagsString=a  ID=bus662  Vbase=400000  Vref=1  Vangle=0  VLF=1  angleLF=0
      settings: AttributesFormatString=|
      | %<ID>
      | %<Vbase>V
      | %<VLF>pu
      | %<angleLF>deg.
      | %<Name>
  bus663 : powerlib/Measurements/Load Flow Bus  LConnTagsString=a  ID=bus663  Vbase=400000  Vref=1  Vangle=0  VLF=1  angleLF=0
      settings: AttributesFormatString=|
      | %<ID>
      | %<Vbase>V
      | %<VLF>pu
      | %<angleLF>deg.
      | %<Name>
  bus664 : powerlib/Measurements/Load Flow Bus  LConnTagsString=a  ID=bus664  Vbase=400000  Vref=1  Vangle=0  VLF=1  angleLF=0
      settings: AttributesFormatString=|
      | %<ID>
      | %<Vbase>V
      | %<VLF>pu
      | %<angleLF>deg.
      | %<Name>
  bus665 : powerlib/Measurements/Load Flow Bus  LConnTagsString=a  ID=bus665  Vbase=400000  Vref=1  Vangle=0  VLF=1  angleLF=0
      settings: AttributesFormatString=|
      | %<ID>
      | %<Vbase>V
      | %<VLF>pu
      | %<angleLF>deg.
      | %<Name>
  bus666 : powerlib/Measurements/Load Flow Bus  LConnTagsString=a  ID=bus666  Vbase=400000  Vref=1  Vangle=0  VLF=1  angleLF=0
      settings: AttributesFormatString=|
      | %<ID>
      | %<Vbase>V
      | %<VLF>pu
      | %<angleLF>deg.
      | %<Name>
  bus667 : powerlib/Measurements/Load Flow Bus  LConnTagsString=a  ID=bus667  Vbase=400000  Vref=1  Vangle=0  VLF=1  angleLF=0
      settings: AttributesFormatString=|
      | %<ID>
      | %<Vbase>V
      | %<VLF>pu
      | %<angleLF>deg.
      | %<Name>
  bus668 : powerlib/Measurements/Load Flow Bus  LConnTagsString=a  ID=bus668  Vbase=400000  Vref=1  Vangle=0  VLF=1  angleLF=0
      settings: AttributesFormatString=|
      | %<ID>
      | %<Vbase>V
      | %<VLF>pu
      | %<angleLF>deg.
      | %<Name>
  bus669 : powerlib/Measurements/Load Flow Bus  LConnTagsString=a  ID=bus669  Vbase=400000  Vref=1  Vangle=0  VLF=1  angleLF=0
      settings: AttributesFormatString=|
      | %<ID>
      | %<Vbase>V
      | %<VLF>pu
      | %<angleLF>deg.
      | %<Name>
  bus67 : powerlib/Measurements/Load Flow Bus  LConnTagsString=a  ID=bus67  Vbase=132000  Vref=1  Vangle=0  VLF=1  angleLF=0
      settings: AttributesFormatString=|
      | %<ID>
      | %<Vbase>V
      | %<VLF>pu
      | %<angleLF>deg.
      | %<Name>
  bus670 : powerlib/Measurements/Load Flow Bus  LConnTagsString=a  ID=bus670  Vbase=400000  Vref=1  Vangle=0  VLF=1  angleLF=0
      settings: AttributesFormatString=|
      | %<ID>
      | %<Vbase>V
      | %<VLF>pu
      | %<angleLF>deg.
      | %<Name>
  bus671 : powerlib/Measurements/Load Flow Bus  LConnTagsString=a  ID=bus671  Vbase=400000  Vref=1  Vangle=0  VLF=1  angleLF=0
      settings: AttributesFormatString=|
      | %<ID>
      | %<Vbase>V
      | %<VLF>pu
      | %<angleLF>deg.
      | %<Name>
  bus672 : powerlib/Measurements/Load Flow Bus  LConnTagsString=a  ID=bus672  Vbase=400000  Vref=1  Vangle=0  VLF=1  angleLF=0
      settings: AttributesFormatString=|
      | %<ID>
      | %<Vbase>V
      | %<VLF>pu
      | %<angleLF>deg.
      | %<Name>
  bus673 : powerlib/Measurements/Load Flow Bus  LConnTagsString=a  ID=bus673  Vbase=400000  Vref=1  Vangle=0  VLF=1  angleLF=0
      settings: AttributesFormatString=|
      | %<ID>
      | %<Vbase>V
      | %<VLF>pu
      | %<angleLF>deg.
      | %<Name>
  bus674 : powerlib/Measurements/Load Flow Bus  LConnTagsString=a  ID=bus674  Vbase=400000  Vref=1  Vangle=0  VLF=1  angleLF=0
      settings: AttributesFormatString=|
      | %<ID>
      | %<Vbase>V
      | %<VLF>pu
      | %<angleLF>deg.
      | %<Name>
  bus675 : powerlib/Measurements/Load Flow Bus  LConnTagsString=a  ID=bus675  Vbase=400000  Vref=1  Vangle=0  VLF=1  angleLF=0
      settings: AttributesFormatString=|
      | %<ID>
      | %<Vbase>V
      | %<VLF>pu
      | %<angleLF>deg.
      | %<Name>
  bus676 : powerlib/Measurements/Load Flow Bus  LConnTagsString=a  ID=bus676  Vbase=400000  Vref=1  Vangle=0  VLF=1  angleLF=0
      settings: AttributesFormatString=|
      | %<ID>
      | %<Vbase>V
      | %<VLF>pu
      | %<angleLF>deg.
      | %<Name>
  bus677 : powerlib/Measurements/Load Flow Bus  LConnTagsString=a  ID=bus677  Vbase=400000  Vref=1  Vangle=0  VLF=1  angleLF=0
      settings: AttributesFormatString=|
      | %<ID>
      | %<Vbase>V
      | %<VLF>pu
      | %<angleLF>deg.
      | %<Name>
  bus678 : powerlib/Measurements/Load Flow Bus  LConnTagsString=a  ID=bus678  Vbase=400000  Vref=1  Vangle=0  VLF=1  angleLF=0
      settings: AttributesFormatString=|
      | %<ID>
      | %<Vbase>V
      | %<VLF>pu
      | %<angleLF>deg.
      | %<Name>
  bus679 : powerlib/Measurements/Load Flow Bus  LConnTagsString=a  ID=bus679  Vbase=400000  Vref=1  Vangle=0  VLF=1  angleLF=0
      settings: AttributesFormatString=|
      | %<ID>
      | %<Vbase>V
      | %<VLF>pu
      | %<angleLF>deg.
      | %<Name>
  bus68 : powerlib/Measurements/Load Flow Bus  LConnTagsString=a  ID=bus68  Vbase=132000  Vref=1  Vangle=0  VLF=1  angleLF=0
      settings: AttributesFormatString=|
      | %<ID>
      | %<Vbase>V
      | %<VLF>pu
      | %<angleLF>deg.
      | %<Name>
  bus680 : powerlib/Measurements/Load Flow Bus  LConnTagsString=a  ID=bus680  Vbase=400000  Vref=1  Vangle=0  VLF=1  angleLF=0
      settings: AttributesFormatString=|
      | %<ID>
      | %<Vbase>V
      | %<VLF>pu
      | %<angleLF>deg.
      | %<Name>
  bus681 : powerlib/Measurements/Load Flow Bus  LConnTagsString=a  ID=bus681  Vbase=400000  Vref=1  Vangle=0  VLF=1  angleLF=0
      settings: AttributesFormatString=|
      | %<ID>
      | %<Vbase>V
      | %<VLF>pu
      | %<angleLF>deg.
      | %<Name>
  bus682 : powerlib/Measurements/Load Flow Bus  LConnTagsString=a  ID=bus682  Vbase=400000  Vref=1  Vangle=0  VLF=1  angleLF=0
      settings: AttributesFormatString=|
      | %<ID>
      | %<Vbase>V
      | %<VLF>pu
      | %<angleLF>deg.
      | %<Name>
  bus683 : powerlib/Measurements/Load Flow Bus  LConnTagsString=a  ID=bus683  Vbase=400000  Vref=1  Vangle=0  VLF=1  angleLF=0
      settings: AttributesFormatString=|
      | %<ID>
      | %<Vbase>V
      | %<VLF>pu
      | %<angleLF>deg.
      | %<Name>
  bus684 : powerlib/Measurements/Load Flow Bus  LConnTagsString=a  ID=bus684  Vbase=400000  Vref=1  Vangle=0  VLF=1  angleLF=0
      settings: AttributesFormatString=|
      | %<ID>
      | %<Vbase>V
      | %<VLF>pu
      | %<angleLF>deg.
      | %<Name>
  bus685 : powerlib/Measurements/Load Flow Bus  LConnTagsString=a  ID=bus685  Vbase=400000  Vref=1  Vangle=0  VLF=1  angleLF=0
      settings: AttributesFormatString=|
      | %<ID>
      | %<Vbase>V
      | %<VLF>pu
      | %<angleLF>deg.
      | %<Name>
  bus69 : powerlib/Measurements/Load Flow Bus  LConnTagsString=a  ID=bus69  Vbase=132000  Vref=1  Vangle=0  VLF=1  angleLF=0
      settings: AttributesFormatString=|
      | %<ID>
      | %<Vbase>V
      | %<VLF>pu
      | %<angleLF>deg.
      | %<Name>
  bus7 : powerlib/Measurements/Load Flow Bus  LConnTagsString=a  ID=bus7  Vbase=132000  Vref=1  Vangle=0  VLF=1  angleLF=0
      settings: AttributesFormatString=|
      | %<ID>
      | %<Vbase>V
      | %<VLF>pu
      | %<angleLF>deg.
      | %<Name>
  bus70 : powerlib/Measurements/Load Flow Bus  LConnTagsString=a  ID=bus70  Vbase=132000  Vref=1  Vangle=0  VLF=1  angleLF=0
      settings: AttributesFormatString=|
      | %<ID>
      | %<Vbase>V
      | %<VLF>pu
      | %<angleLF>deg.
      | %<Name>
  bus71 : powerlib/Measurements/Load Flow Bus  LConnTagsString=a  ID=bus71  Vbase=132000  Vref=1  Vangle=0  VLF=1  angleLF=0
      settings: AttributesFormatString=|
      | %<ID>
      | %<Vbase>V
      | %<VLF>pu
      | %<angleLF>deg.
      | %<Name>
  bus72 : powerlib/Measurements/Load Flow Bus  LConnTagsString=a  ID=bus72  Vbase=132000  Vref=1  Vangle=0  VLF=1  angleLF=0
      settings: AttributesFormatString=|
      | %<ID>
      | %<Vbase>V
      | %<VLF>pu
      | %<angleLF>deg.
      | %<Name>
  bus73 : powerlib/Measurements/Load Flow Bus  LConnTagsString=a  ID=bus73  Vbase=132000  Vref=1  Vangle=0  VLF=1  angleLF=0
      settings: AttributesFormatString=|
      | %<ID>
      | %<Vbase>V
      | %<VLF>pu
      | %<angleLF>deg.
      | %<Name>
  bus74 : powerlib/Measurements/Load Flow Bus  LConnTagsString=a  ID=bus74  Vbase=132000  Vref=1  Vangle=0  VLF=1  angleLF=0
      settings: AttributesFormatString=|
      | %<ID>
      | %<Vbase>V
      | %<VLF>pu
      | %<angleLF>deg.
      | %<Name>
  bus75 : powerlib/Measurements/Load Flow Bus  LConnTagsString=a  ID=bus75  Vbase=132000  Vref=1  Vangle=0  VLF=1  angleLF=0
      settings: AttributesFormatString=|
      | %<ID>
      | %<Vbase>V
      | %<VLF>pu
      | %<angleLF>deg.
      | %<Name>
  bus76 : powerlib/Measurements/Load Flow Bus  LConnTagsString=a  ID=bus76  Vbase=132000  Vref=1  Vangle=0  VLF=1  angleLF=0
      settings: AttributesFormatString=|
      | %<ID>
      | %<Vbase>V
      | %<VLF>pu
      | %<angleLF>deg.
      | %<Name>
  bus77 : powerlib/Measurements/Load Flow Bus  LConnTagsString=a  ID=bus77  Vbase=132000  Vref=1  Vangle=0  VLF=1  angleLF=0
      settings: AttributesFormatString=|
      | %<ID>
      | %<Vbase>V
      | %<VLF>pu
      | %<angleLF>deg.
      | %<Name>
  bus78 : powerlib/Measurements/Load Flow Bus  LConnTagsString=a  ID=bus78  Vbase=132000  Vref=1  Vangle=0  VLF=1  angleLF=0
      settings: AttributesFormatString=|
      | %<ID>
      | %<Vbase>V
      | %<VLF>pu
      | %<angleLF>deg.
      | %<Name>
  bus79 : powerlib/Measurements/Load Flow Bus  LConnTagsString=a  ID=bus79  Vbase=132000  Vref=1  Vangle=0  VLF=1  angleLF=0
      settings: AttributesFormatString=|
      | %<ID>
      | %<Vbase>V
      | %<VLF>pu
      | %<angleLF>deg.
      | %<Name>
  bus8 : powerlib/Measurements/Load Flow Bus  LConnTagsString=a  ID=bus8  Vbase=132000  Vref=1  Vangle=0  VLF=1  angleLF=0
      settings: AttributesFormatString=|
      | %<ID>
      | %<Vbase>V
      | %<VLF>pu
      | %<angleLF>deg.
      | %<Name>
  bus80 : powerlib/Measurements/Load Flow Bus  LConnTagsString=a  ID=bus80  Vbase=132000  Vref=1  Vangle=0  VLF=1  angleLF=0
      settings: AttributesFormatString=|
      | %<ID>
      | %<Vbase>V
      | %<VLF>pu
      | %<angleLF>deg.
      | %<Name>
  bus81 : powerlib/Measurements/Load Flow Bus  LConnTagsString=a  ID=bus81  Vbase=132000  Vref=1  Vangle=0  VLF=1  angleLF=0
      settings: AttributesFormatString=|
      | %<ID>
      | %<Vbase>V
      | %<VLF>pu
      | %<angleLF>deg.
      | %<Name>
  bus82 : powerlib/Measurements/Load Flow Bus  LConnTagsString=a  ID=bus82  Vbase=132000  Vref=1  Vangle=0  VLF=1  angleLF=0
      settings: AttributesFormatString=|
      | %<ID>
      | %<Vbase>V
      | %<VLF>pu
      | %<angleLF>deg.
      | %<Name>
  bus83 : powerlib/Measurements/Load Flow Bus  LConnTagsString=a  ID=bus83  Vbase=132000  Vref=1  Vangle=0  VLF=1  angleLF=0
      settings: AttributesFormatString=|
      | %<ID>
      | %<Vbase>V
      | %<VLF>pu
      | %<angleLF>deg.
      | %<Name>
  bus84 : powerlib/Measurements/Load Flow Bus  LConnTagsString=a  ID=bus84  Vbase=132000  Vref=1  Vangle=0  VLF=1  angleLF=0
      settings: AttributesFormatString=|
      | %<ID>
      | %<Vbase>V
      | %<VLF>pu
      | %<angleLF>deg.
      | %<Name>
  bus85 : powerlib/Measurements/Load Flow Bus  LConnTagsString=a  ID=bus85  Vbase=132000  Vref=1  Vangle=0  VLF=1  angleLF=0
      settings: AttributesFormatString=|
      | %<ID>
      | %<Vbase>V
      | %<VLF>pu
      | %<angleLF>deg.
      | %<Name>
  bus86 : powerlib/Measurements/Load Flow Bus  LConnTagsString=a  ID=bus86  Vbase=132000  Vref=1  Vangle=0  VLF=1  angleLF=0
      settings: AttributesFormatString=|
      | %<ID>
      | %<Vbase>V
      | %<VLF>pu
      | %<angleLF>deg.
      | %<Name>
  bus87 : powerlib/Measurements/Load Flow Bus  LConnTagsString=a  ID=bus87  Vbase=132000  Vref=1  Vangle=0  VLF=1  angleLF=0
      settings: AttributesFormatString=|
      | %<ID>
      | %<Vbase>V
      | %<VLF>pu
      | %<angleLF>deg.
      | %<Name>
  bus88 : powerlib/Measurements/Load Flow Bus  LConnTagsString=a  ID=bus88  Vbase=132000  Vref=1  Vangle=0  VLF=1  angleLF=0
      settings: AttributesFormatString=|
      | %<ID>
      | %<Vbase>V
      | %<VLF>pu
      | %<angleLF>deg.
      | %<Name>
  bus89 : powerlib/Measurements/Load Flow Bus  LConnTagsString=a  ID=bus89  Vbase=132000  Vref=1  Vangle=0  VLF=1  angleLF=0
      settings: AttributesFormatString=|
      | %<ID>
      | %<Vbase>V
      | %<VLF>pu
      | %<angleLF>deg.
      | %<Name>
  bus9 : powerlib/Measurements/Load Flow Bus  LConnTagsString=a  ID=bus9  Vbase=132000  Vref=1  Vangle=0  VLF=1  angleLF=0
      settings: AttributesFormatString=|
      | %<ID>
      | %<Vbase>V
      | %<VLF>pu
      | %<angleLF>deg.
      | %<Name>
  bus90 : powerlib/Measurements/Load Flow Bus  LConnTagsString=a  ID=bus90  Vbase=132000  Vref=1  Vangle=0  VLF=1  angleLF=0
      settings: AttributesFormatString=|
      | %<ID>
      | %<Vbase>V
      | %<VLF>pu
      | %<angleLF>deg.
      | %<Name>
  bus91 : powerlib/Measurements/Load Flow Bus  LConnTagsString=a  ID=bus91  Vbase=132000  Vref=1  Vangle=0  VLF=1  angleLF=0
      settings: AttributesFormatString=|
      | %<ID>
      | %<Vbase>V
      | %<VLF>pu
      | %<angleLF>deg.
      | %<Name>
  bus92 : powerlib/Measurements/Load Flow Bus  LConnTagsString=a  ID=bus92  Vbase=132000  Vref=1  Vangle=0  VLF=1  angleLF=0
      settings: AttributesFormatString=|
      | %<ID>
      | %<Vbase>V
      | %<VLF>pu
      | %<angleLF>deg.
      | %<Name>
  bus93 : powerlib/Measurements/Load Flow Bus  LConnTagsString=a  ID=bus93  Vbase=132000  Vref=1  Vangle=0  VLF=1  angleLF=0
      settings: AttributesFormatString=|
      | %<ID>
      | %<Vbase>V
      | %<VLF>pu
      | %<angleLF>deg.
      | %<Name>
  bus94 : powerlib/Measurements/Load Flow Bus  LConnTagsString=a  ID=bus94  Vbase=132000  Vref=1  Vangle=0  VLF=1  angleLF=0
      settings: AttributesFormatString=|
      | %<ID>
      | %<Vbase>V
      | %<VLF>pu
      | %<angleLF>deg.
      | %<Name>
  bus95 : powerlib/Measurements/Load Flow Bus  LConnTagsString=a  ID=bus95  Vbase=132000  Vref=1  Vangle=0  VLF=1  angleLF=0
      settings: AttributesFormatString=|
      | %<ID>
      | %<Vbase>V
      | %<VLF>pu
      | %<angleLF>deg.
      | %<Name>
  bus96 : powerlib/Measurements/Load Flow Bus  LConnTagsString=a  ID=bus96  Vbase=132000  Vref=1  Vangle=0  VLF=1  angleLF=0
      settings: AttributesFormatString=|
      | %<ID>
      | %<Vbase>V
      | %<VLF>pu
      | %<angleLF>deg.
      | %<Name>
  bus97 : powerlib/Measurements/Load Flow Bus  LConnTagsString=a  ID=bus97  Vbase=132000  Vref=1  Vangle=0  VLF=1  angleLF=0
      settings: AttributesFormatString=|
      | %<ID>
      | %<Vbase>V
      | %<VLF>pu
      | %<angleLF>deg.
      | %<Name>
  bus98 : powerlib/Measurements/Load Flow Bus  LConnTagsString=a  ID=bus98  Vbase=132000  Vref=1  Vangle=0  VLF=1  angleLF=0
      settings: AttributesFormatString=|
      | %<ID>
      | %<Vbase>V
      | %<VLF>pu
      | %<angleLF>deg.
      | %<Name>
  bus99 : powerlib/Measurements/Load Flow Bus  LConnTagsString=a  ID=bus99  Vbase=132000  Vref=1  Vangle=0  VLF=1  angleLF=0
      settings: AttributesFormatString=|
      | %<ID>
      | %<Vbase>V
      | %<VLF>pu
      | %<angleLF>deg.
      | %<Name>
  powergui : powerlib/powergui  Priority=1  SimulationMode=Continuous  SolverType=Tustin  SampleTime=50e-6  frequency=60  SPID=off  DisableSnubberDevices=off  DisableRonSwitches=off  DisableVfSwitches=off  SwTol=0  Interpol=off  DisplayEquations=off  Ts=0  methode=off  frequencyindice=60  Pbase=100e6  ErrMax=1e-4  Iterations=50  UnitsV=kV  UnitsW=MW  FunctionMessages=off  echomessages=off  HookPort=off  EnableUseOfTLC=off  x0status=blocks  RestoreLinks=warning  ResistiveCurrentMeasurement=off  Frange=[0:2:500]  Ylog=off  Xlog=on  ShowGrid=off  save=off  variable=ZData  structure=0  ZoomFFT=off  StartTime=0.0  cycles=1  DisplayStyle=1  fundamental=60  FreqAxis=off  MaxFrequency=1000  frequencyindicesteady=1  RmsSteady=1  display=off
  connections:
  _CN_384824848_132000_CN_115792106_132000/LConn1 -- T_384824848__/LConn1 -- _CN_384824848_132000_CN_239626890_132000/LConn1
  _CN_384824848_132000_CN_115792106_132000/LConn2 -- T_384824848__/LConn2 -- _CN_384824848_132000_CN_239626890_132000/LConn2
  _CN_384824848_132000_CN_115792106_132000/LConn3 -- T_384824848__/LConn3 -- _CN_384824848_132000_CN_239626890_132000/LConn3 -- bus1/LConn1
  _CN_384824848_132000_CN_115792106_132000/RConn1 -- T_115792106__/LConn1 -- _CN_384822726_132000_CN_115792106_132000/LConn1 -- _CN_115717711_132000_CN_115792106_132000/LConn1 -- _CN_239626890_132000_CN_115792106_132000/LConn1
  _CN_384824848_132000_CN_115792106_132000/RConn2 -- T_115792106__/LConn2 -- _CN_384822726_132000_CN_115792106_132000/LConn2 -- _CN_115717711_132000_CN_115792106_132000/LConn2 -- _CN_239626890_132000_CN_115792106_132000/LConn2
  _CN_384824848_132000_CN_115792106_132000/RConn3 -- T_115792106__/LConn3 -- _CN_384822726_132000_CN_115792106_132000/LConn3 -- bus2/LConn1 -- _CN_115717711_132000_CN_115792106_132000/LConn3 -- _CN_239626890_132000_CN_115792106_132000/LConn3
  _CN_384824848_132000_CN_239626890_132000/RConn1 -- T_239626890__/LConn1 -- _CN_239626890_132000_CN_115792106_132000/RConn1 -- _CN_239626890_132000_CN_239581995_132000/LConn1
  _CN_384824848_132000_CN_239626890_132000/RConn2 -- T_239626890__/LConn2 -- _CN_239626890_132000_CN_115792106_132000/RConn2 -- _CN_239626890_132000_CN_239581995_132000/LConn2
  _CN_384824848_132000_CN_239626890_132000/RConn3 -- T_239626890__/LConn3 -- _CN_239626890_132000_CN_115792106_132000/RConn3 -- _CN_239626890_132000_CN_239581995_132000/LConn3 -- bus3/LConn1
  _CN_384752553_132000_CN_239679266_132000/LConn1 -- T_384752553__/LConn1 -- _CN_384752553_132000_CN_384752846_132000/LConn1
  _CN_384752553_132000_CN_239679266_132000/LConn2 -- T_384752553__/LConn2 -- _CN_384752553_132000_CN_384752846_132000/LConn2
  _CN_384752553_132000_CN_239679266_132000/LConn3 -- T_384752553__/LConn3 -- _CN_384752553_132000_CN_384752846_132000/LConn3 -- bus4/LConn1
  _CN_384752553_132000_CN_239679266_132000/RConn1 -- T_239679266__/LConn1 -- _CN_239581995_132000_CN_239679266_132000/LConn1 -- _CN_239679266_132000_CN_239694763_132000/LConn1 -- _CN_239679266_132000_CN_239679334_132000/LConn1 -- _CN_239687287_132000_CN_239679266_132000/LConn1
  _CN_384752553_132000_CN_239679266_132000/RConn2 -- T_239679266__/LConn2 -- _CN_239581995_132000_CN_239679266_132000/LConn2 -- _CN_239679266_132000_CN_239694763_132000/LConn2 -- _CN_239679266_132000_CN_239679334_132000/LConn2 -- _CN_239687287_132000_CN_239679266_132000/LConn2
  _CN_384752553_132000_CN_239679266_132000/RConn3 -- T_239679266__/LConn3 -- _CN_239581995_132000_CN_239679266_132000/LConn3 -- _CN_239679266_132000_CN_239694763_132000/LConn3 -- _CN_239679266_132000_CN_239679334_132000/LConn3 -- bus5/LConn1 -- _CN_239687287_132000_CN_239679266_132000/LConn3
  _CN_384752553_132000_CN_384752846_132000/RConn1 -- T_384752846__/LConn1 -- _CN_384752846_132000_CN_239581995_132000/LConn1 -- _CN_384752846_132000_CN_303315257_132000/LConn1 -- _CN_384752846_132000_CN_303315253_132000/LConn1 -- _CN_242205776_132000_CN_384752846_132000/LConn1 -- _CN_384752846_132000_CN_303315256_132000/LConn1
  _CN_384752553_132000_CN_384752846_132000/RConn2 -- T_384752846__/LConn2 -- _CN_384752846_132000_CN_239581995_132000/LConn2 -- _CN_384752846_132000_CN_303315257_132000/LConn2 -- _CN_384752846_132000_CN_303315253_132000/LConn2 -- _CN_242205776_132000_CN_384752846_132000/LConn2 -- _CN_384752846_132000_CN_303315256_132000/LConn2
  _CN_384752553_132000_CN_384752846_132000/RConn3 -- T_384752846__/LConn3 -- _CN_384752846_132000_CN_239581995_132000/LConn3 -- bus6/LConn1 -- _CN_384752846_132000_CN_303315257_132000/LConn3 -- _CN_384752846_132000_CN_303315253_132000/LConn3 -- _CN_242205776_132000_CN_384752846_132000/LConn3 -- _CN_384752846_132000_CN_303315256_132000/LConn3
  _CN_240050706_132000_CN_240062607_132000/LConn1 -- T_240050706__/LConn1 -- _CN_240050706_132000_CN_240045481_132000/LConn1 -- _CN_240050706_132000_CN_242642583_132000/LConn1
  _CN_240050706_132000_CN_240062607_132000/LConn2 -- T_240050706__/LConn2 -- _CN_240050706_132000_CN_240045481_132000/LConn2 -- _CN_240050706_132000_CN_242642583_132000/LConn2
  _CN_240050706_132000_CN_240062607_132000/LConn3 -- T_240050706__/LConn3 -- _CN_240050706_132000_CN_240045481_132000/LConn3 -- _CN_240050706_132000_CN_242642583_132000/LConn3 -- bus7/LConn1
  _CN_240050706_132000_CN_240062607_132000/RConn1 -- T_240062607__/LConn1 -- _CN_240571747_132000_CN_240062607_132000/LConn1
  _CN_240050706_132000_CN_240062607_132000/RConn2 -- T_240062607__/LConn2 -- _CN_240571747_132000_CN_240062607_132000/LConn2
  _CN_240050706_132000_CN_240062607_132000/RConn3 -- T_240062607__/LConn3 -- _CN_240571747_132000_CN_240062607_132000/LConn3 -- bus8/LConn1
  _CN_240050706_132000_CN_240045481_132000/RConn1 -- T_240045481__/LConn1 -- _CN_239990687_132000_CN_240045481_132000/LConn1 -- _CN_384731081_132000_CN_240045481_132000/LConn1 -- _CN_240000160_132000_CN_240045481_132000/LConn1 -- _CN_242642583_132000_CN_240045481_132000/LConn1
  _CN_240050706_132000_CN_240045481_132000/RConn2 -- T_240045481__/LConn2 -- _CN_239990687_132000_CN_240045481_132000/LConn2 -- _CN_384731081_132000_CN_240045481_132000/LConn2 -- _CN_240000160_132000_CN_240045481_132000/LConn2 -- _CN_242642583_132000_CN_240045481_132000/LConn2
  _CN_240050706_132000_CN_240045481_132000/RConn3 -- T_240045481__/LConn3 -- _CN_239990687_132000_CN_240045481_132000/LConn3 -- _CN_384731081_132000_CN_240045481_132000/LConn3 -- bus9/LConn1 -- _CN_240000160_132000_CN_240045481_132000/LConn3 -- _CN_242642583_132000_CN_240045481_132000/LConn3
  _CN_240050706_132000_CN_242642583_132000/RConn1 -- T_242642583__/LConn1 -- _CN_240000160_132000_CN_242642583_132000/LConn1 -- _CN_242642583_132000_CN_240045481_132000/RConn1
  _CN_240050706_132000_CN_242642583_132000/RConn2 -- T_242642583__/LConn2 -- _CN_240000160_132000_CN_242642583_132000/LConn2 -- _CN_242642583_132000_CN_240045481_132000/RConn2
  _CN_240050706_132000_CN_242642583_132000/RConn3 -- T_242642583__/LConn3 -- _CN_240000160_132000_CN_242642583_132000/LConn3 -- _CN_242642583_132000_CN_240045481_132000/RConn3 -- bus10/LConn1
  T_384800789__/LConn1 -- _CN_384800789_132000_CN_115717271_132000/LConn1
  T_384800789__/LConn2 -- _CN_384800789_132000_CN_115717271_132000/LConn2
  _CN_384800789_132000_CN_115717271_132000/LConn3 -- T_384800789__/LConn3 -- bus11/LConn1
  _CN_384800789_132000_CN_115717271_132000/RConn1 -- T_115717271__/LConn1 -- _CN_115717271_132000_CN_115717276_132000/LConn1
  _CN_384800789_132000_CN_115717271_132000/RConn2 -- T_115717271__/LConn2 -- _CN_115717271_132000_CN_115717276_132000/LConn2
  _CN_384800789_132000_CN_115717271_132000/RConn3 -- T_115717271__/LConn3 -- _CN_115717271_132000_CN_115717276_132000/LConn3 -- bus12/LConn1
  T_203617303__/LConn1 -- _CN_203617303_132000_CN_203615053_132000/LConn1
  T_203617303__/LConn2 -- _CN_203617303_132000_CN_203615053_132000/LConn2
  _CN_203617303_132000_CN_203615053_132000/LConn3 -- T_203617303__/LConn3 -- bus13/LConn1
  T_203615053__/LConn1 -- _CN_203617303_132000_CN_203615053_132000/RConn1
  T_203615053__/LConn2 -- _CN_203617303_132000_CN_203615053_132000/RConn2
  _CN_203617303_132000_CN_203615053_132000/RConn3 -- T_203615053__/LConn3 -- bus14/LConn1
  T_29499934__/LConn1 -- _CN_29499934_132000_CN_354619026_132000/LConn1
  T_29499934__/LConn2 -- _CN_29499934_132000_CN_354619026_132000/LConn2
  _CN_29499934_132000_CN_354619026_132000/LConn3 -- T_29499934__/LConn3 -- bus15/LConn1
  _CN_29499934_132000_CN_354619026_132000/RConn1 -- T_354619026__/LConn1 -- _CN_384961291_132000_CN_354619026_132000/LConn1 -- _CN_354619026_132000_CN_181332756_132000/LConn1
  _CN_29499934_132000_CN_354619026_132000/RConn2 -- T_354619026__/LConn2 -- _CN_384961291_132000_CN_354619026_132000/LConn2 -- _CN_354619026_132000_CN_181332756_132000/LConn2
  _CN_29499934_132000_CN_354619026_132000/RConn3 -- T_354619026__/LConn3 -- _CN_384961291_132000_CN_354619026_132000/LConn3 -- _CN_354619026_132000_CN_181332756_132000/LConn3 -- bus16/LConn1
  T_176665128__Substation_Kalba/LConn1 -- _CN_176665128_132000_CN_220817213_132000/LConn1
  T_176665128__Substation_Kalba/LConn2 -- _CN_176665128_132000_CN_220817213_132000/LConn2
  _CN_176665128_132000_CN_220817213_132000/LConn3 -- T_176665128__Substation_Kalba/LConn3 -- bus17/LConn1
  _CN_176665128_132000_CN_220817213_132000/RConn1 -- T_220817213__substation_Al_Hayl/LConn1 -- _CN_260963603_132000_CN_220817213_132000/LConn1
  _CN_176665128_132000_CN_220817213_132000/RConn2 -- T_220817213__substation_Al_Hayl/LConn2 -- _CN_260963603_132000_CN_220817213_132000/LConn2
  _CN_176665128_132000_CN_220817213_132000/RConn3 -- T_220817213__substation_Al_Hayl/LConn3 -- _CN_260963603_132000_CN_220817213_132000/LConn3 -- bus18/LConn1
  T_115205161__/LConn1 -- _CN_115205161_132000_CN_52609391_132000/LConn1
  T_115205161__/LConn2 -- _CN_115205161_132000_CN_52609391_132000/LConn2
  _CN_115205161_132000_CN_52609391_132000/LConn3 -- T_115205161__/LConn3 -- bus19/LConn1
  _CN_115205161_132000_CN_52609391_132000/RConn1 -- T_52609391__/LConn1 -- _CN_115188435_132000_CN_52609391_132000/LConn1
  _CN_115205161_132000_CN_52609391_132000/RConn2 -- T_52609391__/LConn2 -- _CN_115188435_132000_CN_52609391_132000/LConn2
  _CN_115205161_132000_CN_52609391_132000/RConn3 -- T_52609391__/LConn3 -- _CN_115188435_132000_CN_52609391_132000/LConn3 -- bus20/LConn1
  _CN_375782442_132000_CN_386056423_132000/LConn1 -- T_375782442__/LConn1 -- _CN_375782442_132000_CN_386056422_132000/LConn1
  _CN_375782442_132000_CN_386056423_132000/LConn2 -- T_375782442__/LConn2 -- _CN_375782442_132000_CN_386056422_132000/LConn2
  _CN_375782442_132000_CN_386056423_132000/LConn3 -- T_375782442__/LConn3 -- _CN_375782442_132000_CN_386056422_132000/LConn3 -- bus21/LConn1
  _CN_375782442_132000_CN_386056423_132000/RConn1 -- T_386056423__/LConn1 -- _CN_94816849_132000_CN_386056423_132000/LConn1
  _CN_375782442_132000_CN_386056423_132000/RConn2 -- T_386056423__/LConn2 -- _CN_94816849_132000_CN_386056423_132000/LConn2
  _CN_375782442_132000_CN_386056423_132000/RConn3 -- T_386056423__/LConn3 -- _CN_94816849_132000_CN_386056423_132000/LConn3 -- bus22/LConn1
  _CN_375782442_132000_CN_386056422_132000/RConn1 -- T_386056422__/LConn1 -- _CN_94816849_132000_CN_386056422_132000/LConn1
  _CN_375782442_132000_CN_386056422_132000/RConn2 -- T_386056422__/LConn2 -- _CN_94816849_132000_CN_386056422_132000/LConn2
  _CN_375782442_132000_CN_386056422_132000/RConn3 -- T_386056422__/LConn3 -- _CN_94816849_132000_CN_386056422_132000/LConn3 -- bus23/LConn1
  _CN_232335918_132000_CN_223140233_132000/LConn1 -- T_232335918__/LConn1 -- _CN_232335918_132000_CN_39657769_132000/LConn1
  _CN_232335918_132000_CN_223140233_132000/LConn2 -- T_232335918__/LConn2 -- _CN_232335918_132000_CN_39657769_132000/LConn2
  _CN_232335918_132000_CN_223140233_132000/LConn3 -- T_232335918__/LConn3 -- _CN_232335918_132000_CN_39657769_132000/LConn3 -- bus24/LConn1
  _CN_232335918_132000_CN_223140233_132000/RConn1 -- T_223140233__/LConn1 -- _CN_115717711_132000_CN_223140233_132000/LConn1 -- _CN_115717269_132000_CN_223140233_132000/LConn1
  _CN_232335918_132000_CN_223140233_132000/RConn2 -- T_223140233__/LConn2 -- _CN_115717711_132000_CN_223140233_132000/LConn2 -- _CN_115717269_132000_CN_223140233_132000/LConn2
  _CN_232335918_132000_CN_223140233_132000/RConn3 -- T_223140233__/LConn3 -- _CN_115717711_132000_CN_223140233_132000/LConn3 -- _CN_115717269_132000_CN_223140233_132000/LConn3 -- bus25/LConn1
  _CN_232335918_132000_CN_39657769_132000/RConn1 -- T_39657769__/LConn1 -- _CN_39657769_132000_CN_115677372_132000/LConn1
  _CN_232335918_132000_CN_39657769_132000/RConn2 -- T_39657769__/LConn2 -- _CN_39657769_132000_CN_115677372_132000/LConn2
  _CN_232335918_132000_CN_39657769_132000/RConn3 -- T_39657769__/LConn3 -- _CN_39657769_132000_CN_115677372_132000/LConn3 -- bus26/LConn1
  T_384714801__/LConn1 -- _CN_384714801_132000_CN_384714800_132000/LConn1
  T_384714801__/LConn2 -- _CN_384714801_132000_CN_384714800_132000/LConn2
  _CN_384714801_132000_CN_384714800_132000/LConn3 -- T_384714801__/LConn3 -- bus27/LConn1
  _CN_384714801_132000_CN_384714800_132000/RConn1 -- G_384714800_/RConn1 -- _CN_384714810_132000_CN_384714800_132000/LConn1
  _CN_384714801_132000_CN_384714800_132000/RConn2 -- G_384714800_/RConn2 -- _CN_384714810_132000_CN_384714800_132000/LConn2
  _CN_384714801_132000_CN_384714800_132000/RConn3 -- G_384714800_/RConn3 -- _CN_384714810_132000_CN_384714800_132000/LConn3 -- bus28/LConn1
  _CN_386214966_132000_CN_385548908_132000/LConn1 -- T_386214966__/LConn1 -- _CN_386214966_132000_CN_60333463_132000/LConn1
  _CN_386214966_132000_CN_385548908_132000/LConn2 -- T_386214966__/LConn2 -- _CN_386214966_132000_CN_60333463_132000/LConn2
  _CN_386214966_132000_CN_385548908_132000/LConn3 -- T_386214966__/LConn3 -- _CN_386214966_132000_CN_60333463_132000/LConn3 -- bus29/LConn1
  _CN_386214966_132000_CN_385548908_132000/RConn1 -- T_385548908__/LConn1 -- _CN_385548908_132000_CN_354672637_132000/LConn1 -- _CN_385548908_132000_CN_115677372_132000/LConn1
  _CN_386214966_132000_CN_385548908_132000/RConn2 -- T_385548908__/LConn2 -- _CN_385548908_132000_CN_354672637_132000/LConn2 -- _CN_385548908_132000_CN_115677372_132000/LConn2
  _CN_386214966_132000_CN_385548908_132000/RConn3 -- T_385548908__/LConn3 -- _CN_385548908_132000_CN_354672637_132000/LConn3 -- bus30/LConn1 -- _CN_385548908_132000_CN_115677372_132000/LConn3
  T_60333463__/LConn1 -- _CN_386214966_132000_CN_60333463_132000/RConn1
  T_60333463__/LConn2 -- _CN_386214966_132000_CN_60333463_132000/RConn2
  _CN_386214966_132000_CN_60333463_132000/RConn3 -- T_60333463__/LConn3 -- bus31/LConn1
  T_384714810__/LConn1 -- _CN_384714810_132000_CN_384714800_132000/RConn1
  T_384714810__/LConn2 -- _CN_384714810_132000_CN_384714800_132000/RConn2
  _CN_384714810_132000_CN_384714800_132000/RConn3 -- T_384714810__/LConn3 -- bus32/LConn1
  _CN_385907829_132000_CN_29495157_132000/LConn1 -- T_385907829__/LConn1 -- _CN_385907829_132000_CN_385907824_132000/LConn1 -- _CN_385907829_132000_CN_173271221_132000/LConn1
  _CN_385907829_132000_CN_29495157_132000/LConn2 -- T_385907829__/LConn2 -- _CN_385907829_132000_CN_385907824_132000/LConn2 -- _CN_385907829_132000_CN_173271221_132000/LConn2
  _CN_385907829_132000_CN_29495157_132000/LConn3 -- T_385907829__/LConn3 -- _CN_385907829_132000_CN_385907824_132000/LConn3 -- _CN_385907829_132000_CN_173271221_132000/LConn3 -- bus33/LConn1
  _CN_385907829_132000_CN_29495157_132000/RConn1 -- T_29495157__/RConn1 -- _CN_385907825_132000_CN_29495157_132000/LConn1 -- L_29495157/LConn1
  _CN_385907829_132000_CN_29495157_132000/RConn2 -- T_29495157__/RConn2 -- _CN_385907825_132000_CN_29495157_132000/LConn2 -- L_29495157/LConn2
  _CN_385907829_132000_CN_29495157_132000/RConn3 -- T_29495157__/RConn3 -- _CN_385907825_132000_CN_29495157_132000/LConn3 -- L_29495157/LConn3 -- bus34/LConn1
  T_385907824__/LConn1 -- _CN_385907829_132000_CN_385907824_132000/RConn1
  T_385907824__/LConn2 -- _CN_385907829_132000_CN_385907824_132000/RConn2
  _CN_385907829_132000_CN_385907824_132000/RConn3 -- T_385907824__/LConn3 -- bus35/LConn1
  T_173271221__/LConn1 -- _CN_385907829_132000_CN_173271221_132000/RConn1
  T_173271221__/LConn2 -- _CN_385907829_132000_CN_173271221_132000/RConn2
  _CN_385907829_132000_CN_173271221_132000/RConn3 -- T_173271221__/LConn3 -- bus36/LConn1
  T_384714812__/LConn1 -- _CN_384714812_132000_CN_240571747_132000/LConn1
  T_384714812__/LConn2 -- _CN_384714812_132000_CN_240571747_132000/LConn2
  _CN_384714812_132000_CN_240571747_132000/LConn3 -- T_384714812__/LConn3 -- bus37/LConn1
  _CN_384714812_132000_CN_240571747_132000/RConn1 -- T_240571747__/LConn1 -- _CN_240571747_132000_CN_240571748_132000/LConn1 -- _CN_240571747_132000_CN_240062607_132000/RConn1
  _CN_384714812_132000_CN_240571747_132000/RConn2 -- T_240571747__/LConn2 -- _CN_240571747_132000_CN_240571748_132000/LConn2 -- _CN_240571747_132000_CN_240062607_132000/RConn2
  _CN_384714812_132000_CN_240571747_132000/RConn3 -- T_240571747__/LConn3 -- _CN_240571747_132000_CN_240571748_132000/LConn3 -- _CN_240571747_132000_CN_240062607_132000/RConn3 -- bus38/LConn1
  T_203985985__/LConn1 -- _CN_203985985_132000_CN_203888070_132000/LConn1
  T_203985985__/LConn2 -- _CN_203985985_132000_CN_203888070_132000/LConn2
  _CN_203985985_132000_CN_203888070_132000/LConn3 -- T_203985985__/LConn3 -- bus39/LConn1
  T_203888070__/LConn1 -- _CN_203985985_132000_CN_203888070_132000/RConn1
  T_203888070__/LConn2 -- _CN_203985985_132000_CN_203888070_132000/RConn2
  _CN_203985985_132000_CN_203888070_132000/RConn3 -- T_203888070__/LConn3 -- bus40/LConn1
  _CN_384961291_132000_CN_354619026_132000/RConn1 -- T_384961291__/LConn1 -- _CN_384961291_132000_CN_94816858_132000/LConn1 -- _CN_384961291_132000_CN_384961303_132000/LConn1 -- _CN_384961291_132000_CN_384961300_132000/LConn1
  _CN_384961291_132000_CN_354619026_132000/RConn2 -- T_384961291__/LConn2 -- _CN_384961291_132000_CN_94816858_132000/LConn2 -- _CN_384961291_132000_CN_384961303_132000/LConn2 -- _CN_384961291_132000_CN_384961300_132000/LConn2
  _CN_384961291_132000_CN_354619026_132000/RConn3 -- T_384961291__/LConn3 -- _CN_384961291_132000_CN_94816858_132000/LConn3 -- _CN_384961291_132000_CN_384961303_132000/LConn3 -- _CN_384961291_132000_CN_384961300_132000/LConn3 -- bus41/LConn1
  _CN_384961291_132000_CN_94816858_132000/RConn1 -- T_94816858__/LConn1 -- _CN_94816858_132000_CN_146511548_132000/LConn1
  _CN_384961291_132000_CN_94816858_132000/RConn2 -- T_94816858__/LConn2 -- _CN_94816858_132000_CN_146511548_132000/LConn2
  _CN_384961291_132000_CN_94816858_132000/RConn3 -- T_94816858__/LConn3 -- _CN_94816858_132000_CN_146511548_132000/LConn3 -- bus42/LConn1
  _CN_384961291_132000_CN_384961303_132000/RConn1 -- T_384961303__/LConn1 -- _CN_384961303_132000_CN_379753822_132000/LConn1
  _CN_384961291_132000_CN_384961303_132000/RConn2 -- T_384961303__/LConn2 -- _CN_384961303_132000_CN_379753822_132000/LConn2
  _CN_384961291_132000_CN_384961303_132000/RConn3 -- T_384961303__/LConn3 -- _CN_384961303_132000_CN_379753822_132000/LConn3 -- bus43/LConn1
  _CN_384961291_132000_CN_384961300_132000/RConn1 -- T_384961300__/LConn1 -- _CN_384961300_132000_CN_94816975_132000/LConn1
  _CN_384961291_132000_CN_384961300_132000/RConn2 -- T_384961300__/LConn2 -- _CN_384961300_132000_CN_94816975_132000/LConn2
  _CN_384961291_132000_CN_384961300_132000/RConn3 -- T_384961300__/LConn3 -- _CN_384961300_132000_CN_94816975_132000/LConn3 -- bus44/LConn1
  _CN_328560711_132000_CN_123775127_132000/LConn1 -- T_328560711__/LConn1 -- _CN_328560711_132000_CN_168770199_132000/LConn1
  _CN_328560711_132000_CN_123775127_132000/LConn2 -- T_328560711__/LConn2 -- _CN_328560711_132000_CN_168770199_132000/LConn2
  _CN_328560711_132000_CN_123775127_132000/LConn3 -- T_328560711__/LConn3 -- _CN_328560711_132000_CN_168770199_132000/LConn3 -- bus45/LConn1
  T_123775127__/LConn1 -- _CN_328560711_132000_CN_123775127_132000/RConn1
  T_123775127__/LConn2 -- _CN_328560711_132000_CN_123775127_132000/RConn2
  _CN_328560711_132000_CN_123775127_132000/RConn3 -- T_123775127__/LConn3 -- bus46/LConn1
  T_168770199__/LConn1 -- _CN_328560711_132000_CN_168770199_132000/RConn1
  T_168770199__/LConn2 -- _CN_328560711_132000_CN_168770199_132000/RConn2
  _CN_328560711_132000_CN_168770199_132000/RConn3 -- T_168770199__/LConn3 -- bus47/LConn1
  _CN_132132424_132000_CN_132154026_132000/LConn1 -- T_132132424__/LConn1 -- _CN_132132424_132000_CN_112321201_132000/LConn1 -- _CN_132132424_132000_CN_112521127_132000/LConn1
  _CN_132132424_132000_CN_132154026_132000/LConn2 -- T_132132424__/LConn2 -- _CN_132132424_132000_CN_112321201_132000/LConn2 -- _CN_132132424_132000_CN_112521127_132000/LConn2
  _CN_132132424_132000_CN_132154026_132000/LConn3 -- T_132132424__/LConn3 -- _CN_132132424_132000_CN_112321201_132000/LConn3 -- _CN_132132424_132000_CN_112521127_132000/LConn3 -- bus48/LConn1
  T_132154026__/LConn1 -- _CN_132132424_132000_CN_132154026_132000/RConn1
  T_132154026__/LConn2 -- _CN_132132424_132000_CN_132154026_132000/RConn2
  _CN_132132424_132000_CN_132154026_132000/RConn3 -- T_132154026__/LConn3 -- bus49/LConn1
  _CN_132132424_132000_CN_112321201_132000/RConn1 -- T_112321201__substation/LConn1 -- _CN_112460404_132000_CN_112321201_132000/LConn1
  _CN_132132424_132000_CN_112321201_132000/RConn2 -- T_112321201__substation/LConn2 -- _CN_112460404_132000_CN_112321201_132000/LConn2
  _CN_132132424_132000_CN_112321201_132000/RConn3 -- T_112321201__substation/LConn3 -- _CN_112460404_132000_CN_112321201_132000/LConn3 -- bus50/LConn1
  T_112521127__substation/LConn1 -- _CN_132132424_132000_CN_112521127_132000/RConn1
  T_112521127__substation/LConn2 -- _CN_132132424_132000_CN_112521127_132000/RConn2
  _CN_132132424_132000_CN_112521127_132000/RConn3 -- T_112521127__substation/LConn3 -- bus51/LConn1
  T_122262836__/LConn1 -- _CN_122262836_132000_CN_121847629_132000/LConn1
  T_122262836__/LConn2 -- _CN_122262836_132000_CN_121847629_132000/LConn2
  _CN_122262836_132000_CN_121847629_132000/LConn3 -- T_122262836__/LConn3 -- bus52/LConn1
  _CN_122262836_132000_CN_121847629_132000/RConn1 -- T_121847629__/RConn1 -- _CN_121847629_132000_CN_181133259_132000/LConn1 -- L_121847629/LConn1
  _CN_122262836_132000_CN_121847629_132000/RConn2 -- T_121847629__/RConn2 -- _CN_121847629_132000_CN_181133259_132000/LConn2 -- L_121847629/LConn2
  _CN_122262836_132000_CN_121847629_132000/RConn3 -- T_121847629__/RConn3 -- _CN_121847629_132000_CN_181133259_132000/LConn3 -- L_121847629/LConn3 -- bus53/LConn1
  _CN_239976013_132000_CN_239939959_132000/LConn1 -- T_239976013__/LConn1 -- _CN_239976013_132000_CN_239937124_132000/LConn1 -- _CN_239976013_132000_CN_384684174_132000/LConn1
  _CN_239976013_132000_CN_239939959_132000/LConn2 -- T_239976013__/LConn2 -- _CN_239976013_132000_CN_239937124_132000/LConn2 -- _CN_239976013_132000_CN_384684174_132000/LConn2
  _CN_239976013_132000_CN_239939959_132000/LConn3 -- T_239976013__/LConn3 -- _CN_239976013_132000_CN_239937124_132000/LConn3 -- _CN_239976013_132000_CN_384684174_132000/LConn3 -- bus54/LConn1
  _CN_239976013_132000_CN_239939959_132000/RConn1 -- T_239939959__/LConn1 -- _CN_239937124_132000_CN_239939959_132000/LConn1
  _CN_239976013_132000_CN_239939959_132000/RConn2 -- T_239939959__/LConn2 -- _CN_239937124_132000_CN_239939959_132000/LConn2
  _CN_239976013_132000_CN_239939959_132000/RConn3 -- T_239939959__/LConn3 -- _CN_239937124_132000_CN_239939959_132000/LConn3 -- bus55/LConn1
  _CN_239976013_132000_CN_239937124_132000/RConn1 -- T_239937124__/LConn1 -- _CN_239937124_132000_CN_242539627_132000/LConn1 -- _CN_239937124_132000_CN_239435500_132000/LConn1 -- _CN_239937124_132000_CN_239939959_132000/RConn1
  _CN_239976013_132000_CN_239937124_132000/RConn2 -- T_239937124__/LConn2 -- _CN_239937124_132000_CN_242539627_132000/LConn2 -- _CN_239937124_132000_CN_239435500_132000/LConn2 -- _CN_239937124_132000_CN_239939959_132000/RConn2
  _CN_239976013_132000_CN_239937124_132000/RConn3 -- T_239937124__/LConn3 -- _CN_239937124_132000_CN_242539627_132000/LConn3 -- _CN_239937124_132000_CN_239435500_132000/LConn3 -- _CN_239937124_132000_CN_239939959_132000/RConn3 -- bus56/LConn1
  _CN_239976013_132000_CN_384684174_132000/RConn1 -- T_384684174__/LConn1 -- _CN_384684174_132000_CN_239990697_132000/LConn1
  _CN_239976013_132000_CN_384684174_132000/RConn2 -- T_384684174__/LConn2 -- _CN_384684174_132000_CN_239990697_132000/LConn2
  _CN_239976013_132000_CN_384684174_132000/RConn3 -- T_384684174__/LConn3 -- _CN_384684174_132000_CN_239990697_132000/LConn3 -- bus57/LConn1
  _CN_115717711_132000_CN_115792106_132000/RConn1 -- T_115717711__/LConn1 -- _CN_115717711_132000_CN_115797297_132000/LConn1 -- _CN_115717711_132000_CN_115797291_132000/LConn1 -- _CN_115717711_132000_CN_223140233_132000/RConn1 -- _CN_115717711_132000_CN_115792105_132000/LConn1
  _CN_115717711_132000_CN_115792106_132000/RConn2 -- T_115717711__/LConn2 -- _CN_115717711_132000_CN_115797297_132000/LConn2 -- _CN_115717711_132000_CN_115797291_132000/LConn2 -- _CN_115717711_132000_CN_223140233_132000/RConn2 -- _CN_115717711_132000_CN_115792105_132000/LConn2
  _CN_115717711_132000_CN_115792106_132000/RConn3 -- T_115717711__/LConn3 -- _CN_115717711_132000_CN_115797297_132000/LConn3 -- _CN_115717711_132000_CN_115797291_132000/LConn3 -- bus58/LConn1 -- _CN_115717711_132000_CN_223140233_132000/RConn3 -- _CN_115717711_132000_CN_115792105_132000/LConn3
  _CN_115717711_132000_CN_115792105_132000/RConn1 -- G_115792105_/RConn1 -- _CN_384908661_132000_CN_115792105_132000/LConn1
  _CN_115717711_132000_CN_115792105_132000/RConn2 -- G_115792105_/RConn2 -- _CN_384908661_132000_CN_115792105_132000/LConn2
  _CN_115717711_132000_CN_115792105_132000/RConn3 -- G_115792105_/RConn3 -- _CN_384908661_132000_CN_115792105_132000/LConn3 -- bus59/LConn1
  _CN_115717711_132000_CN_115797297_132000/RConn1 -- T_115797297__/LConn1 -- _CN_115797297_132000_CN_115797300_132000/LConn1
  _CN_115717711_132000_CN_115797297_132000/RConn2 -- T_115797297__/LConn2 -- _CN_115797297_132000_CN_115797300_132000/LConn2
  _CN_115717711_132000_CN_115797297_132000/RConn3 -- T_115797297__/LConn3 -- _CN_115797297_132000_CN_115797300_132000/LConn3 -- bus60/LConn1
  T_115797291__/LConn1 -- _CN_115717711_132000_CN_115797291_132000/RConn1
  T_115797291__/LConn2 -- _CN_115717711_132000_CN_115797291_132000/RConn2
  _CN_115717711_132000_CN_115797291_132000/RConn3 -- T_115797291__/LConn3 -- bus61/LConn1
  _CN_242205776_132000_CN_242166513_132000/LConn1 -- T_242205776__/LConn1 -- _CN_242205776_132000_CN_239581995_132000/LConn1 -- _CN_242205776_132000_CN_384753595_132000/LConn1 -- _CN_242205776_132000_CN_384911487_132000/LConn1 -- _CN_242205776_132000_CN_353897470_132000/LConn1 -- _CN_242205776_132000_CN_242205780_132000/LConn1 -- _CN_242205776_132000_CN_384752846_132000/RConn1
  _CN_242205776_132000_CN_242166513_132000/LConn2 -- T_242205776__/LConn2 -- _CN_242205776_132000_CN_239581995_132000/LConn2 -- _CN_242205776_132000_CN_384753595_132000/LConn2 -- _CN_242205776_132000_CN_384911487_132000/LConn2 -- _CN_242205776_132000_CN_353897470_132000/LConn2 -- _CN_242205776_132000_CN_242205780_132000/LConn2 -- _CN_242205776_132000_CN_384752846_132000/RConn2
  _CN_242205776_132000_CN_242166513_132000/LConn3 -- T_242205776__/LConn3 -- _CN_242205776_132000_CN_239581995_132000/LConn3 -- _CN_242205776_132000_CN_384753595_132000/LConn3 -- _CN_242205776_132000_CN_384911487_132000/LConn3 -- _CN_242205776_132000_CN_353897470_132000/LConn3 -- _CN_242205776_132000_CN_242205780_132000/LConn3 -- _CN_242205776_132000_CN_384752846_132000/RConn3 -- bus62/LConn1
  _CN_242205776_132000_CN_242166513_132000/RConn1 -- T_242166513__/LConn1 -- _CN_239581995_132000_CN_242166513_132000/LConn1
  _CN_242205776_132000_CN_242166513_132000/RConn2 -- T_242166513__/LConn2 -- _CN_239581995_132000_CN_242166513_132000/LConn2
  _CN_242205776_132000_CN_242166513_132000/RConn3 -- T_242166513__/LConn3 -- _CN_239581995_132000_CN_242166513_132000/LConn3 -- bus63/LConn1
  _CN_242205776_132000_CN_239581995_132000/RConn1 -- T_239581995__/LConn1 -- _CN_239581995_132000_CN_239679266_132000/RConn1 -- _CN_239581995_132000_CN_239581958_132000/LConn1 -- _CN_239581995_132000_CN_242166513_132000/RConn1 -- _CN_239626890_132000_CN_239581995_132000/RConn1 -- _CN_384752846_132000_CN_239581995_132000/RConn1
  _CN_242205776_132000_CN_239581995_132000/RConn2 -- T_239581995__/LConn2 -- _CN_239581995_132000_CN_239679266_132000/RConn2 -- _CN_239581995_132000_CN_239581958_132000/LConn2 -- _CN_239581995_132000_CN_242166513_132000/RConn2 -- _CN_239626890_132000_CN_239581995_132000/RConn2 -- _CN_384752846_132000_CN_239581995_132000/RConn2
  _CN_242205776_132000_CN_239581995_132000/RConn3 -- T_239581995__/LConn3 -- _CN_239581995_132000_CN_239679266_132000/RConn3 -- bus64/LConn1 -- _CN_239581995_132000_CN_239581958_132000/LConn3 -- _CN_239581995_132000_CN_242166513_132000/RConn3 -- _CN_239626890_132000_CN_239581995_132000/RConn3 -- _CN_384752846_132000_CN_239581995_132000/RConn3
  T_384753595__/LConn1 -- _CN_242205776_132000_CN_384753595_132000/RConn1
  T_384753595__/LConn2 -- _CN_242205776_132000_CN_384753595_132000/RConn2
  _CN_242205776_132000_CN_384753595_132000/RConn3 -- T_384753595__/LConn3 -- bus65/LConn1
  T_384911487__/LConn1 -- _CN_242205776_132000_CN_384911487_132000/RConn1
  T_384911487__/LConn2 -- _CN_242205776_132000_CN_384911487_132000/RConn2
  _CN_242205776_132000_CN_384911487_132000/RConn3 -- T_384911487__/LConn3 -- bus66/LConn1
  T_353897470__/LConn1 -- _CN_242205776_132000_CN_353897470_132000/RConn1
  T_353897470__/LConn2 -- _CN_242205776_132000_CN_353897470_132000/RConn2
  _CN_242205776_132000_CN_353897470_132000/RConn3 -- T_353897470__/LConn3 -- bus67/LConn1
  T_242205780__/LConn1 -- _CN_242205776_132000_CN_242205780_132000/RConn1
  T_242205780__/LConn2 -- _CN_242205776_132000_CN_242205780_132000/RConn2
  _CN_242205776_132000_CN_242205780_132000/RConn3 -- T_242205780__/LConn3 -- bus68/LConn1
  _CN_94816849_132000_CN_386056423_132000/RConn1 -- T_94816849__/LConn1 -- _CN_94816849_132000_CN_181332831_132000/LConn1 -- _CN_94816849_132000_CN_386056422_132000/RConn1
  _CN_94816849_132000_CN_386056423_132000/RConn2 -- T_94816849__/LConn2 -- _CN_94816849_132000_CN_181332831_132000/LConn2 -- _CN_94816849_132000_CN_386056422_132000/RConn2
  _CN_94816849_132000_CN_386056423_132000/RConn3 -- T_94816849__/LConn3 -- _CN_94816849_132000_CN_181332831_132000/LConn3 -- bus69/LConn1 -- _CN_94816849_132000_CN_386056422_132000/RConn3
  T_181332831__/LConn1 -- _CN_94816849_132000_CN_181332831_132000/RConn1
  T_181332831__/LConn2 -- _CN_94816849_132000_CN_181332831_132000/RConn2
  _CN_94816849_132000_CN_181332831_132000/RConn3 -- T_181332831__/LConn3 -- bus70/LConn1
  T_240571748__/LConn1 -- _CN_240571747_132000_CN_240571748_132000/RConn1
  T_240571748__/LConn2 -- _CN_240571747_132000_CN_240571748_132000/RConn2
  _CN_240571747_132000_CN_240571748_132000/RConn3 -- T_240571748__/LConn3 -- bus71/LConn1
  _CN_204266069_132000_CN_204267684_132000/LConn1 -- T_204266069__/LConn1 -- _CN_204266069_132000_CN_204553547_132000/LConn1
  _CN_204266069_132000_CN_204267684_132000/LConn2 -- T_204266069__/LConn2 -- _CN_204266069_132000_CN_204553547_132000/LConn2
  _CN_204266069_132000_CN_204267684_132000/LConn3 -- T_204266069__/LConn3 -- _CN_204266069_132000_CN_204553547_132000/LConn3 -- bus72/LConn1
  _CN_204266069_132000_CN_204267684_132000/RConn1 -- T_204267684__/LConn1 -- _CN_204267684_132000_CN_204142303_132000/LConn1
  _CN_204266069_132000_CN_204267684_132000/RConn2 -- T_204267684__/LConn2 -- _CN_204267684_132000_CN_204142303_132000/LConn2
  _CN_204266069_132000_CN_204267684_132000/RConn3 -- T_204267684__/LConn3 -- _CN_204267684_132000_CN_204142303_132000/LConn3 -- bus73/LConn1
  T_204553547__substation/LConn1 -- _CN_204266069_132000_CN_204553547_132000/RConn1
  T_204553547__substation/LConn2 -- _CN_204266069_132000_CN_204553547_132000/RConn2
  _CN_204266069_132000_CN_204553547_132000/RConn3 -- T_204553547__substation/LConn3 -- bus74/LConn1
  T_146511548__/LConn1 -- _CN_94816858_132000_CN_146511548_132000/RConn1
  T_146511548__/LConn2 -- _CN_94816858_132000_CN_146511548_132000/RConn2
  _CN_94816858_132000_CN_146511548_132000/RConn3 -- T_146511548__/LConn3 -- bus75/LConn1
  _CN_239937124_132000_CN_242539627_132000/RConn1 -- T_242539627__/LConn1 -- _CN_242539627_132000_CN_239435500_132000/LConn1 -- _CN_242539627_132000_CN_384708869_132000/LConn1 -- _CN_242539627_132000_CN_239946325_132000/LConn1
  _CN_239937124_132000_CN_242539627_132000/RConn2 -- T_242539627__/LConn2 -- _CN_242539627_132000_CN_239435500_132000/LConn2 -- _CN_242539627_132000_CN_384708869_132000/LConn2 -- _CN_242539627_132000_CN_239946325_132000/LConn2
  _CN_239937124_132000_CN_242539627_132000/RConn3 -- T_242539627__/LConn3 -- _CN_242539627_132000_CN_239435500_132000/LConn3 -- _CN_242539627_132000_CN_384708869_132000/LConn3 -- _CN_242539627_132000_CN_239946325_132000/LConn3 -- bus76/LConn1
  _CN_239937124_132000_CN_239435500_132000/RConn1 -- T_239435500__/LConn1 -- _CN_242539627_132000_CN_239435500_132000/RConn1 -- _CN_242544315_132000_CN_239435500_132000/LConn1 -- _CN_239435500_132000_CN_239435499_132000/LConn1
  _CN_239937124_132000_CN_239435500_132000/RConn2 -- T_239435500__/LConn2 -- _CN_242539627_132000_CN_239435500_132000/RConn2 -- _CN_242544315_132000_CN_239435500_132000/LConn2 -- _CN_239435500_132000_CN_239435499_132000/LConn2
  _CN_239937124_132000_CN_239435500_132000/RConn3 -- T_239435500__/LConn3 -- _CN_242539627_132000_CN_239435500_132000/RConn3 -- _CN_242544315_132000_CN_239435500_132000/LConn3 -- _CN_239435500_132000_CN_239435499_132000/LConn3 -- bus77/LConn1
  _CN_386200252_132000_CN_354672632_132000/LConn1 -- T_386200252__/LConn1 -- _CN_386200252_132000_CN_60333184_132000/LConn1
  _CN_386200252_132000_CN_354672632_132000/LConn2 -- T_386200252__/LConn2 -- _CN_386200252_132000_CN_60333184_132000/LConn2
  _CN_386200252_132000_CN_354672632_132000/LConn3 -- T_386200252__/LConn3 -- _CN_386200252_132000_CN_60333184_132000/LConn3 -- bus78/LConn1
  _CN_386200252_132000_CN_354672632_132000/RConn1 -- T_354672632__/RConn1 -- _CN_386202923_132000_CN_354672632_132000/LConn1 -- L_354672632/LConn1 -- _CN_386200253_132000_CN_354672632_132000/LConn1
  _CN_386200252_132000_CN_354672632_132000/RConn2 -- T_354672632__/RConn2 -- _CN_386202923_132000_CN_354672632_132000/LConn2 -- L_354672632/LConn2 -- _CN_386200253_132000_CN_354672632_132000/LConn2
  _CN_386200252_132000_CN_354672632_132000/RConn3 -- T_354672632__/RConn3 -- _CN_386202923_132000_CN_354672632_132000/LConn3 -- L_354672632/LConn3 -- bus79/LConn1 -- _CN_386200253_132000_CN_354672632_132000/LConn3
  _CN_386200252_132000_CN_60333184_132000/RConn1 -- T_60333184__/LConn1 -- _CN_60333184_132000_CN_60234385_132000/LConn1 -- _CN_60333184_132000_CN_168549720_132000/LConn1
  _CN_386200252_132000_CN_60333184_132000/RConn2 -- T_60333184__/LConn2 -- _CN_60333184_132000_CN_60234385_132000/LConn2 -- _CN_60333184_132000_CN_168549720_132000/LConn2
  _CN_386200252_132000_CN_60333184_132000/RConn3 -- T_60333184__/LConn3 -- _CN_60333184_132000_CN_60234385_132000/LConn3 -- _CN_60333184_132000_CN_168549720_132000/LConn3 -- bus80/LConn1
  T_384708869__/LConn1 -- _CN_242539627_132000_CN_384708869_132000/RConn1
  T_384708869__/LConn2 -- _CN_242539627_132000_CN_384708869_132000/RConn2
  _CN_242539627_132000_CN_384708869_132000/RConn3 -- T_384708869__/LConn3 -- bus81/LConn1
  _CN_242539627_132000_CN_239946325_132000/RConn1 -- T_239946325__/LConn1 -- _CN_384684166_132000_CN_239946325_132000/LConn1
  _CN_242539627_132000_CN_239946325_132000/RConn2 -- T_239946325__/LConn2 -- _CN_384684166_132000_CN_239946325_132000/LConn2
  _CN_242539627_132000_CN_239946325_132000/RConn3 -- T_239946325__/LConn3 -- _CN_384684166_132000_CN_239946325_132000/LConn3 -- bus82/LConn1
  _CN_385548908_132000_CN_115677372_132000/RConn1 -- G_115677372_/RConn1 -- _CN_39657768_132000_CN_115677372_132000/LConn1 -- _CN_39657769_132000_CN_115677372_132000/RConn1 -- _CN_39657770_132000_CN_115677372_132000/LConn1
  _CN_385548908_132000_CN_115677372_132000/RConn2 -- G_115677372_/RConn2 -- _CN_39657768_132000_CN_115677372_132000/LConn2 -- _CN_39657769_132000_CN_115677372_132000/RConn2 -- _CN_39657770_132000_CN_115677372_132000/LConn2
  _CN_385548908_132000_CN_115677372_132000/RConn3 -- G_115677372_/RConn3 -- _CN_39657768_132000_CN_115677372_132000/LConn3 -- _CN_39657769_132000_CN_115677372_132000/RConn3 -- _CN_39657770_132000_CN_115677372_132000/LConn3 -- bus83/LConn1
  _CN_385548908_132000_CN_354672637_132000/RConn1 -- T_354672637__/LConn1 -- _CN_60234385_132000_CN_354672637_132000/LConn1
  _CN_385548908_132000_CN_354672637_132000/RConn2 -- T_354672637__/LConn2 -- _CN_60234385_132000_CN_354672637_132000/LConn2
  _CN_385548908_132000_CN_354672637_132000/RConn3 -- T_354672637__/LConn3 -- _CN_60234385_132000_CN_354672637_132000/LConn3 -- bus84/LConn1
  _CN_386200253_132000_CN_354672632_132000/RConn1 -- T_386200253__/LConn1 -- _CN_386200253_132000_CN_39657770_132000/LConn1
  _CN_386200253_132000_CN_354672632_132000/RConn2 -- T_386200253__/LConn2 -- _CN_386200253_132000_CN_39657770_132000/LConn2
  _CN_386200253_132000_CN_354672632_132000/RConn3 -- T_386200253__/LConn3 -- _CN_386200253_132000_CN_39657770_132000/LConn3 -- bus85/LConn1
  _CN_386200253_132000_CN_39657770_132000/RConn1 -- T_39657770__/LConn1 -- _CN_39657770_132000_CN_115677372_132000/RConn1
  _CN_386200253_132000_CN_39657770_132000/RConn2 -- T_39657770__/LConn2 -- _CN_39657770_132000_CN_115677372_132000/RConn2
  _CN_386200253_132000_CN_39657770_132000/RConn3 -- T_39657770__/LConn3 -- _CN_39657770_132000_CN_115677372_132000/RConn3 -- bus86/LConn1
  _CN_385907825_132000_CN_385907834_132000/LConn1 -- T_385907825__/LConn1 -- _CN_385907825_132000_CN_29495157_132000/RConn1
  _CN_385907825_132000_CN_385907834_132000/LConn2 -- T_385907825__/LConn2 -- _CN_385907825_132000_CN_29495157_132000/RConn2
  _CN_385907825_132000_CN_385907834_132000/LConn3 -- T_385907825__/LConn3 -- _CN_385907825_132000_CN_29495157_132000/RConn3 -- bus87/LConn1
  T_385907834__/LConn1 -- _CN_385907825_132000_CN_385907834_132000/RConn1
  T_385907834__/LConn2 -- _CN_385907825_132000_CN_385907834_132000/RConn2
  _CN_385907825_132000_CN_385907834_132000/RConn3 -- T_385907834__/LConn3 -- bus88/LConn1
  _CN_384902258_132000_CN_354672633_132000/LConn1 -- T_384902258__/LConn1 -- _CN_384902258_132000_CN_240196788_132000/LConn1 -- _CN_384902258_132000_CN_384902262_132000/LConn1
  _CN_384902258_132000_CN_354672633_132000/LConn2 -- T_384902258__/LConn2 -- _CN_384902258_132000_CN_240196788_132000/LConn2 -- _CN_384902258_132000_CN_384902262_132000/LConn2
  _CN_384902258_132000_CN_354672633_132000/LConn3 -- T_384902258__/LConn3 -- _CN_384902258_132000_CN_240196788_132000/LConn3 -- _CN_384902258_132000_CN_384902262_132000/LConn3 -- bus89/LConn1
  T_354672633__/LConn1 -- _CN_384902258_132000_CN_354672633_132000/RConn1
  T_354672633__/LConn2 -- _CN_384902258_132000_CN_354672633_132000/RConn2
  _CN_384902258_132000_CN_354672633_132000/RConn3 -- T_354672633__/LConn3 -- bus90/LConn1
  T_240196788__/LConn1 -- _CN_384902258_132000_CN_240196788_132000/RConn1
  T_240196788__/LConn2 -- _CN_384902258_132000_CN_240196788_132000/RConn2
  _CN_384902258_132000_CN_240196788_132000/RConn3 -- T_240196788__/LConn3 -- bus91/LConn1
  T_384902262__/LConn1 -- _CN_384902258_132000_CN_384902262_132000/RConn1
  T_384902262__/LConn2 -- _CN_384902258_132000_CN_384902262_132000/RConn2
  _CN_384902258_132000_CN_384902262_132000/RConn3 -- T_384902262__/LConn3 -- bus92/LConn1
  _CN_112460404_132000_CN_295186316_132000/LConn1 -- T_112460404__/LConn1 -- _CN_112460404_132000_CN_112460405_132000/LConn1 -- _CN_112460404_132000_CN_112321201_132000/RConn1
  _CN_112460404_132000_CN_295186316_132000/LConn2 -- T_112460404__/LConn2 -- _CN_112460404_132000_CN_112460405_132000/LConn2 -- _CN_112460404_132000_CN_112321201_132000/RConn2
  _CN_112460404_132000_CN_295186316_132000/LConn3 -- T_112460404__/LConn3 -- _CN_112460404_132000_CN_112460405_132000/LConn3 -- _CN_112460404_132000_CN_112321201_132000/RConn3 -- bus93/LConn1
  T_295186316__/LConn1 -- _CN_112460404_132000_CN_295186316_132000/RConn1
  T_295186316__/LConn2 -- _CN_112460404_132000_CN_295186316_132000/RConn2
  _CN_112460404_132000_CN_295186316_132000/RConn3 -- T_295186316__/LConn3 -- bus94/LConn1
  T_112460405__/LConn1 -- _CN_112460404_132000_CN_112460405_132000/RConn1
  T_112460405__/LConn2 -- _CN_112460404_132000_CN_112460405_132000/RConn2
  _CN_112460404_132000_CN_112460405_132000/RConn3 -- T_112460405__/LConn3 -- bus95/LConn1
  T_199776373__/LConn1 -- _CN_199776373_132000_CN_181132741_132000/LConn1
  T_199776373__/LConn2 -- _CN_199776373_132000_CN_181132741_132000/LConn2
  _CN_199776373_132000_CN_181132741_132000/LConn3 -- T_199776373__/LConn3 -- bus96/LConn1
  _CN_199776373_132000_CN_181132741_132000/RConn1 -- T_181132741__/RConn1 -- _CN_168190854_132000_CN_181132741_132000/LConn1 -- _CN_181132699_132000_CN_181132741_132000/LConn1 -- L_181132741/LConn1
  _CN_199776373_132000_CN_181132741_132000/RConn2 -- T_181132741__/RConn2 -- _CN_168190854_132000_CN_181132741_132000/LConn2 -- _CN_181132699_132000_CN_181132741_132000/LConn2 -- L_181132741/LConn2
  _CN_199776373_132000_CN_181132741_132000/RConn3 -- T_181132741__/RConn3 -- _CN_168190854_132000_CN_181132741_132000/LConn3 -- _CN_181132699_132000_CN_181132741_132000/LConn3 -- L_181132741/LConn3 -- bus97/LConn1
  _CN_239687287_132000_CN_239694763_132000/LConn1 -- T_239687287__/LConn1 -- _CN_239687287_132000_CN_239679266_132000/RConn1
  _CN_239687287_132000_CN_239694763_132000/LConn2 -- T_239687287__/LConn2 -- _CN_239687287_132000_CN_239679266_132000/RConn2
  _CN_239687287_132000_CN_239694763_132000/LConn3 -- T_239687287__/LConn3 -- _CN_239687287_132000_CN_239679266_132000/RConn3 -- bus98/LConn1
  _CN_239687287_132000_CN_239694763_132000/RConn1 -- T_239694763__/LConn1 -- _CN_243443456_132000_CN_239694763_132000/LConn1 -- _CN_239679266_132000_CN_239694763_132000/RConn1 -- _CN_242544315_132000_CN_239694763_132000/LConn1
  _CN_239687287_132000_CN_239694763_132000/RConn2 -- T_239694763__/LConn2 -- _CN_243443456_132000_CN_239694763_132000/LConn2 -- _CN_239679266_132000_CN_239694763_132000/RConn2 -- _CN_242544315_132000_CN_239694763_132000/LConn2
  _CN_239687287_132000_CN_239694763_132000/RConn3 -- T_239694763__/LConn3 -- _CN_243443456_132000_CN_239694763_132000/LConn3 -- _CN_239679266_132000_CN_239694763_132000/RConn3 -- bus99/LConn1 -- _CN_242544315_132000_CN_239694763_132000/LConn3
  T_223684728__/LConn1 -- _CN_223684728_132000_CN_379753822_132000/LConn1
  T_223684728__/LConn2 -- _CN_223684728_132000_CN_379753822_132000/LConn2
  _CN_223684728_132000_CN_379753822_132000/LConn3 -- T_223684728__/LConn3 -- bus100/LConn1
  _CN_223684728_132000_CN_379753822_132000/RConn1 -- T_379753822__/LConn1 -- _CN_384961303_132000_CN_379753822_132000/RConn1
  _CN_223684728_132000_CN_379753822_132000/RConn2 -- T_379753822__/LConn2 -- _CN_384961303_132000_CN_379753822_132000/RConn2
  _CN_223684728_132000_CN_379753822_132000/RConn3 -- T_379753822__/LConn3 -- _CN_384961303_132000_CN_379753822_132000/RConn3 -- bus101/LConn1
  T_424681663__/LConn1 -- _CN_424681663_132000_CN_424681664_132000/LConn1
  T_424681663__/LConn2 -- _CN_424681663_132000_CN_424681664_132000/LConn2
  _CN_424681663_132000_CN_424681664_132000/LConn3 -- T_424681663__/LConn3 -- bus102/LConn1
  _CN_424681663_132000_CN_424681664_132000/RConn1 -- T_424681664__/LConn1 -- _CN_424681664_132000_CN_201082863_132000/LConn1 -- _CN_424681664_132000_CN_424681656_132000/LConn1
  _CN_424681663_132000_CN_424681664_132000/RConn2 -- T_424681664__/LConn2 -- _CN_424681664_132000_CN_201082863_132000/LConn2 -- _CN_424681664_132000_CN_424681656_132000/LConn2
  _CN_424681663_132000_CN_424681664_132000/RConn3 -- T_424681664__/LConn3 -- _CN_424681664_132000_CN_201082863_132000/LConn3 -- bus103/LConn1 -- _CN_424681664_132000_CN_424681656_132000/LConn3
  _CN_60333184_132000_CN_60234385_132000/RConn1 -- T_60234385__/RConn1 -- _CN_60234385_132000_CN_263373386_132000/LConn1 -- _CN_60234385_132000_CN_354672637_132000/RConn1 -- _CN_60234385_132000_CN_115677406_132000/LConn1 -- L_60234385/LConn1
  _CN_60333184_132000_CN_60234385_132000/RConn2 -- T_60234385__/RConn2 -- _CN_60234385_132000_CN_263373386_132000/LConn2 -- _CN_60234385_132000_CN_354672637_132000/RConn2 -- _CN_60234385_132000_CN_115677406_132000/LConn2 -- L_60234385/LConn2
  _CN_60333184_132000_CN_60234385_132000/RConn3 -- T_60234385__/RConn3 -- _CN_60234385_132000_CN_263373386_132000/LConn3 -- _CN_60234385_132000_CN_354672637_132000/RConn3 -- _CN_60234385_132000_CN_115677406_132000/LConn3 -- L_60234385/LConn3 -- bus104/LConn1
  T_168549720__/LConn1 -- _CN_60333184_132000_CN_168549720_132000/RConn1
  T_168549720__/LConn2 -- _CN_60333184_132000_CN_168549720_132000/RConn2
  _CN_60333184_132000_CN_168549720_132000/RConn3 -- T_168549720__/LConn3 -- bus105/LConn1
  _CN_385113219_132000_CN_227922803_132000/LConn1 -- T_385113219__/LConn1 -- _CN_385113219_132000_CN_94816976_132000/LConn1
  _CN_385113219_132000_CN_227922803_132000/LConn2 -- T_385113219__/LConn2 -- _CN_385113219_132000_CN_94816976_132000/LConn2
  _CN_385113219_132000_CN_227922803_132000/LConn3 -- T_385113219__/LConn3 -- _CN_385113219_132000_CN_94816976_132000/LConn3 -- bus106/LConn1
  _CN_385113219_132000_CN_227922803_132000/RConn1 -- T_227922803__/LConn1 -- _CN_94816976_132000_CN_227922803_132000/LConn1
  _CN_385113219_132000_CN_227922803_132000/RConn2 -- T_227922803__/LConn2 -- _CN_94816976_132000_CN_227922803_132000/LConn2
  _CN_385113219_132000_CN_227922803_132000/RConn3 -- T_227922803__/LConn3 -- _CN_94816976_132000_CN_227922803_132000/LConn3 -- bus107/LConn1
  _CN_385113219_132000_CN_94816976_132000/RConn1 -- T_94816976__/LConn1 -- _CN_385113202_132000_CN_94816976_132000/LConn1 -- _CN_94816976_132000_CN_173919914_132000/LConn1 -- _CN_94816976_132000_CN_227922803_132000/RConn1
  _CN_385113219_132000_CN_94816976_132000/RConn2 -- T_94816976__/LConn2 -- _CN_385113202_132000_CN_94816976_132000/LConn2 -- _CN_94816976_132000_CN_173919914_132000/LConn2 -- _CN_94816976_132000_CN_227922803_132000/RConn2
  _CN_385113219_132000_CN_94816976_132000/RConn3 -- T_94816976__/LConn3 -- _CN_385113202_132000_CN_94816976_132000/LConn3 -- _CN_94816976_132000_CN_173919914_132000/LConn3 -- _CN_94816976_132000_CN_227922803_132000/RConn3 -- bus108/LConn1
  _CN_384684166_132000_CN_239990687_132000/LConn1 -- T_384684166__/LConn1 -- _CN_384684166_132000_CN_239990697_132000/LConn1 -- _CN_384684166_132000_CN_239946325_132000/RConn1 -- _CN_384684166_132000_CN_240000160_132000/LConn1
  _CN_384684166_132000_CN_239990687_132000/LConn2 -- T_384684166__/LConn2 -- _CN_384684166_132000_CN_239990697_132000/LConn2 -- _CN_384684166_132000_CN_239946325_132000/RConn2 -- _CN_384684166_132000_CN_240000160_132000/LConn2
  _CN_384684166_132000_CN_239990687_132000/LConn3 -- T_384684166__/LConn3 -- _CN_384684166_132000_CN_239990697_132000/LConn3 -- bus109/LConn1 -- _CN_384684166_132000_CN_239946325_132000/RConn3 -- _CN_384684166_132000_CN_240000160_132000/LConn3
  _CN_384684166_132000_CN_239990687_132000/RConn1 -- T_239990687__/LConn1 -- _CN_239990687_132000_CN_240045481_132000/RConn1
  _CN_384684166_132000_CN_239990687_132000/RConn2 -- T_239990687__/LConn2 -- _CN_239990687_132000_CN_240045481_132000/RConn2
  _CN_384684166_132000_CN_239990687_132000/RConn3 -- T_239990687__/LConn3 -- _CN_239990687_132000_CN_240045481_132000/RConn3 -- bus110/LConn1
  _CN_384684166_132000_CN_240000160_132000/RConn1 -- T_240000160__/LConn1 -- _CN_240000160_132000_CN_240045481_132000/RConn1 -- _CN_240000160_132000_CN_242642583_132000/RConn1
  _CN_384684166_132000_CN_240000160_132000/RConn2 -- T_240000160__/LConn2 -- _CN_240000160_132000_CN_240045481_132000/RConn2 -- _CN_240000160_132000_CN_242642583_132000/RConn2
  _CN_384684166_132000_CN_240000160_132000/RConn3 -- T_240000160__/LConn3 -- _CN_240000160_132000_CN_240045481_132000/RConn3 -- _CN_240000160_132000_CN_242642583_132000/RConn3 -- bus111/LConn1
  _CN_384684166_132000_CN_239990697_132000/RConn1 -- T_239990697__/LConn1 -- _CN_384684174_132000_CN_239990697_132000/RConn1 -- _CN_384688538_132000_CN_239990697_132000/LConn1 -- _CN_239990697_132000_CN_384688544_132000/LConn1
  _CN_384684166_132000_CN_239990697_132000/RConn2 -- T_239990697__/LConn2 -- _CN_384684174_132000_CN_239990697_132000/RConn2 -- _CN_384688538_132000_CN_239990697_132000/LConn2 -- _CN_239990697_132000_CN_384688544_132000/LConn2
  _CN_384684166_132000_CN_239990697_132000/RConn3 -- T_239990697__/LConn3 -- _CN_384684174_132000_CN_239990697_132000/RConn3 -- _CN_384688538_132000_CN_239990697_132000/LConn3 -- _CN_239990697_132000_CN_384688544_132000/LConn3 -- bus112/LConn1
  G_263373386_/RConn1 -- _CN_60234385_132000_CN_263373386_132000/RConn1
  G_263373386_/RConn2 -- _CN_60234385_132000_CN_263373386_132000/RConn2
  _CN_60234385_132000_CN_263373386_132000/RConn3 -- G_263373386_/RConn3 -- bus113/LConn1
  T_115677406__/LConn1 -- _CN_60234385_132000_CN_115677406_132000/RConn1
  T_115677406__/LConn2 -- _CN_60234385_132000_CN_115677406_132000/RConn2
  _CN_60234385_132000_CN_115677406_132000/RConn3 -- T_115677406__/LConn3 -- bus114/LConn1
  _CN_354619026_132000_CN_181332756_132000/RConn1 -- T_181332756__/RConn4 -- _CN_260963603_132000_CN_181332756_132000/LConn1 -- L_181332756/LConn1 -- _CN_181332751_132000_CN_181332756_132000/LConn1
  _CN_354619026_132000_CN_181332756_132000/RConn2 -- T_181332756__/RConn5 -- _CN_260963603_132000_CN_181332756_132000/LConn2 -- L_181332756/LConn2 -- _CN_181332751_132000_CN_181332756_132000/LConn2
  _CN_354619026_132000_CN_181332756_132000/RConn3 -- T_181332756__/RConn6 -- _CN_260963603_132000_CN_181332756_132000/LConn3 -- L_181332756/LConn3 -- bus115/LConn1 -- _CN_181332751_132000_CN_181332756_132000/LConn3
  T_384908661__/LConn1 -- _CN_384908661_132000_CN_115792105_132000/RConn1
  T_384908661__/LConn2 -- _CN_384908661_132000_CN_115792105_132000/RConn2
  _CN_384908661_132000_CN_115792105_132000/RConn3 -- T_384908661__/LConn3 -- bus116/LConn1
  T_115717268__/LConn1 -- _CN_115717268_132000_CN_115717276_132000/LConn1
  T_115717268__/LConn2 -- _CN_115717268_132000_CN_115717276_132000/LConn2
  _CN_115717268_132000_CN_115717276_132000/LConn3 -- T_115717268__/LConn3 -- bus117/LConn1
  _CN_115717268_132000_CN_115717276_132000/RConn1 -- T_115717276__/LConn1 -- _CN_115717275_132000_CN_115717276_132000/LConn1 -- _CN_115717276_132000_CN_115717277_132000/LConn1 -- _CN_115717271_132000_CN_115717276_132000/RConn1
  _CN_115717268_132000_CN_115717276_132000/RConn2 -- T_115717276__/LConn2 -- _CN_115717275_132000_CN_115717276_132000/LConn2 -- _CN_115717276_132000_CN_115717277_132000/LConn2 -- _CN_115717271_132000_CN_115717276_132000/RConn2
  _CN_115717268_132000_CN_115717276_132000/RConn3 -- T_115717276__/LConn3 -- _CN_115717275_132000_CN_115717276_132000/LConn3 -- _CN_115717276_132000_CN_115717277_132000/LConn3 -- bus118/LConn1 -- _CN_115717271_132000_CN_115717276_132000/RConn3
  _CN_115717269_132000_CN_115717275_132000/LConn1 -- T_115717269__/LConn1 -- _CN_115717269_132000_CN_223140233_132000/RConn1
  _CN_115717269_132000_CN_115717275_132000/LConn2 -- T_115717269__/LConn2 -- _CN_115717269_132000_CN_223140233_132000/RConn2
  _CN_115717269_132000_CN_115717275_132000/LConn3 -- T_115717269__/LConn3 -- _CN_115717269_132000_CN_223140233_132000/RConn3 -- bus119/LConn1
  _CN_115717269_132000_CN_115717275_132000/RConn1 -- T_115717275__/LConn1 -- _CN_115717275_132000_CN_115717276_132000/RConn1
  _CN_115717269_132000_CN_115717275_132000/RConn2 -- T_115717275__/LConn2 -- _CN_115717275_132000_CN_115717276_132000/RConn2
  _CN_115717269_132000_CN_115717275_132000/RConn3 -- T_115717275__/LConn3 -- _CN_115717275_132000_CN_115717276_132000/RConn3 -- bus120/LConn1
  T_189281434__/LConn1 -- _CN_189281434_132000_CN_168190854_132000/LConn1
  T_189281434__/LConn2 -- _CN_189281434_132000_CN_168190854_132000/LConn2
  _CN_189281434_132000_CN_168190854_132000/LConn3 -- T_189281434__/LConn3 -- bus121/LConn1
  _CN_189281434_132000_CN_168190854_132000/RConn1 -- T_168190854__/LConn1 -- _CN_168190854_132000_CN_181132741_132000/RConn1
  _CN_189281434_132000_CN_168190854_132000/RConn2 -- T_168190854__/LConn2 -- _CN_168190854_132000_CN_181132741_132000/RConn2
  _CN_189281434_132000_CN_168190854_132000/RConn3 -- T_168190854__/LConn3 -- _CN_168190854_132000_CN_181132741_132000/RConn3 -- bus122/LConn1
  G_115717277_/RConn1 -- _CN_115717276_132000_CN_115717277_132000/RConn1
  G_115717277_/RConn2 -- _CN_115717276_132000_CN_115717277_132000/RConn2
  _CN_115717276_132000_CN_115717277_132000/RConn3 -- G_115717277_/RConn3 -- bus123/LConn1
  T_94816929__/LConn1 -- _CN_94816929_132000_CN_173919914_132000/LConn1
  T_94816929__/LConn2 -- _CN_94816929_132000_CN_173919914_132000/LConn2
  _CN_94816929_132000_CN_173919914_132000/LConn3 -- T_94816929__/LConn3 -- bus124/LConn1
  _CN_94816929_132000_CN_173919914_132000/RConn1 -- T_173919914__/LConn1 -- _CN_94816976_132000_CN_173919914_132000/RConn1
  _CN_94816929_132000_CN_173919914_132000/RConn2 -- T_173919914__/LConn2 -- _CN_94816976_132000_CN_173919914_132000/RConn2
  _CN_94816929_132000_CN_173919914_132000/RConn3 -- T_173919914__/LConn3 -- _CN_94816976_132000_CN_173919914_132000/RConn3 -- bus125/LConn1
  _CN_204267684_132000_CN_204142303_132000/RConn1 -- T_204142303__/LConn1 -- _CN_204142303_132000_CN_204141035_132000/LConn1
  _CN_204267684_132000_CN_204142303_132000/RConn2 -- T_204142303__/LConn2 -- _CN_204142303_132000_CN_204141035_132000/LConn2
  _CN_204267684_132000_CN_204142303_132000/RConn3 -- T_204142303__/LConn3 -- _CN_204142303_132000_CN_204141035_132000/LConn3 -- bus126/LConn1
  _CN_301911494_132000_CN_385263258_132000/LConn1 -- T_301911494__/RConn1 -- L_301911494/LConn1
  _CN_301911494_132000_CN_385263258_132000/LConn2 -- T_301911494__/RConn2 -- L_301911494/LConn2
  _CN_301911494_132000_CN_385263258_132000/LConn3 -- T_301911494__/RConn3 -- L_301911494/LConn3 -- bus127/LConn1
  _CN_301911494_132000_CN_385263258_132000/RConn1 -- T_385263258__/LConn1 -- _CN_260963603_132000_CN_385263258_132000/LConn1
  _CN_301911494_132000_CN_385263258_132000/RConn2 -- T_385263258__/LConn2 -- _CN_260963603_132000_CN_385263258_132000/LConn2
  _CN_301911494_132000_CN_385263258_132000/RConn3 -- T_385263258__/LConn3 -- _CN_260963603_132000_CN_385263258_132000/LConn3 -- bus128/LConn1
  _CN_298351271_132000_CN_133861049_132000/LConn1 -- T_298351271__/LConn1 -- _CN_298351271_132000_CN_133861050_132000/LConn1 -- _CN_298351271_132000_CN_168862805_132000/LConn1
  _CN_298351271_132000_CN_133861049_132000/LConn2 -- T_298351271__/LConn2 -- _CN_298351271_132000_CN_133861050_132000/LConn2 -- _CN_298351271_132000_CN_168862805_132000/LConn2
  _CN_298351271_132000_CN_133861049_132000/LConn3 -- T_298351271__/LConn3 -- _CN_298351271_132000_CN_133861050_132000/LConn3 -- bus129/LConn1 -- _CN_298351271_132000_CN_168862805_132000/LConn3
  _CN_298351271_132000_CN_133861049_132000/RConn1 -- T_133861049__/LConn1 -- _CN_133861049_132000_CN_133865685_132000/LConn1
  _CN_298351271_132000_CN_133861049_132000/RConn2 -- T_133861049__/LConn2 -- _CN_133861049_132000_CN_133865685_132000/LConn2
  _CN_298351271_132000_CN_133861049_132000/RConn3 -- T_133861049__/LConn3 -- _CN_133861049_132000_CN_133865685_132000/LConn3 -- bus130/LConn1
  G_168862805_/RConn1 -- _CN_298351271_132000_CN_168862805_132000/RConn1
  G_168862805_/RConn2 -- _CN_298351271_132000_CN_168862805_132000/RConn2
  _CN_298351271_132000_CN_168862805_132000/RConn3 -- G_168862805_/RConn3 -- bus131/LConn1
  T_133861050__/LConn1 -- _CN_298351271_132000_CN_133861050_132000/RConn1
  T_133861050__/LConn2 -- _CN_298351271_132000_CN_133861050_132000/RConn2
  _CN_298351271_132000_CN_133861050_132000/RConn3 -- T_133861050__/LConn3 -- bus132/LConn1
  T_384822726__/LConn1 -- _CN_384822726_132000_CN_115792106_132000/RConn1
  T_384822726__/LConn2 -- _CN_384822726_132000_CN_115792106_132000/RConn2
  _CN_384822726_132000_CN_115792106_132000/RConn3 -- T_384822726__/LConn3 -- bus133/LConn1
  _CN_385113202_132000_CN_29499064_132000/LConn1 -- T_385113202__/LConn1 -- _CN_385113202_132000_CN_94816976_132000/RConn1
  _CN_385113202_132000_CN_29499064_132000/LConn2 -- T_385113202__/LConn2 -- _CN_385113202_132000_CN_94816976_132000/RConn2
  _CN_385113202_132000_CN_29499064_132000/LConn3 -- T_385113202__/LConn3 -- _CN_385113202_132000_CN_94816976_132000/RConn3 -- bus134/LConn1
  _CN_385113202_132000_CN_29499064_132000/RConn1 -- T_29499064__/RConn1 -- L_29499064/LConn1
  _CN_385113202_132000_CN_29499064_132000/RConn2 -- T_29499064__/RConn2 -- L_29499064/LConn2
  _CN_385113202_132000_CN_29499064_132000/RConn3 -- T_29499064__/RConn3 -- L_29499064/LConn3 -- bus135/LConn1
  _CN_384961300_132000_CN_94816975_132000/RConn1 -- T_94816975__/LConn1 -- _CN_385086141_132000_CN_94816975_132000/LConn1
  _CN_384961300_132000_CN_94816975_132000/RConn2 -- T_94816975__/LConn2 -- _CN_385086141_132000_CN_94816975_132000/LConn2
  _CN_384961300_132000_CN_94816975_132000/RConn3 -- T_94816975__/LConn3 -- _CN_385086141_132000_CN_94816975_132000/LConn3 -- bus136/LConn1
  T_133865685__/LConn1 -- _CN_133861049_132000_CN_133865685_132000/RConn1
  T_133865685__/LConn2 -- _CN_133861049_132000_CN_133865685_132000/RConn2
  _CN_133861049_132000_CN_133865685_132000/RConn3 -- T_133865685__/LConn3 -- bus137/LConn1
  _CN_242544315_132000_CN_384708877_132000/LConn1 -- T_242544315__/LConn1 -- _CN_242544315_132000_CN_239694763_132000/RConn1 -- _CN_242544315_132000_CN_384708875_132000/LConn1 -- _CN_242544315_132000_CN_239435500_132000/RConn1 -- _CN_242544315_132000_CN_243443456_132000/LConn1
  _CN_242544315_132000_CN_384708877_132000/LConn2 -- T_242544315__/LConn2 -- _CN_242544315_132000_CN_239694763_132000/RConn2 -- _CN_242544315_132000_CN_384708875_132000/LConn2 -- _CN_242544315_132000_CN_239435500_132000/RConn2 -- _CN_242544315_132000_CN_243443456_132000/LConn2
  _CN_242544315_132000_CN_384708877_132000/LConn3 -- T_242544315__/LConn3 -- _CN_242544315_132000_CN_239694763_132000/RConn3 -- _CN_242544315_132000_CN_384708875_132000/LConn3 -- _CN_242544315_132000_CN_239435500_132000/RConn3 -- _CN_242544315_132000_CN_243443456_132000/LConn3 -- bus138/LConn1
  T_384708877__/LConn1 -- _CN_242544315_132000_CN_384708877_132000/RConn1
  T_384708877__/LConn2 -- _CN_242544315_132000_CN_384708877_132000/RConn2
  _CN_242544315_132000_CN_384708877_132000/RConn3 -- T_384708877__/LConn3 -- bus139/LConn1
  T_384708875__/LConn1 -- _CN_242544315_132000_CN_384708875_132000/RConn1
  T_384708875__/LConn2 -- _CN_242544315_132000_CN_384708875_132000/RConn2
  _CN_242544315_132000_CN_384708875_132000/RConn3 -- T_384708875__/LConn3 -- bus140/LConn1
  _CN_242544315_132000_CN_243443456_132000/RConn1 -- T_243443456__/LConn1 -- _CN_243443456_132000_CN_239694763_132000/RConn1
  _CN_242544315_132000_CN_243443456_132000/RConn2 -- T_243443456__/LConn2 -- _CN_243443456_132000_CN_239694763_132000/RConn2
  _CN_242544315_132000_CN_243443456_132000/RConn3 -- T_243443456__/LConn3 -- _CN_243443456_132000_CN_239694763_132000/RConn3 -- bus141/LConn1
  T_385086141__/LConn1 -- _CN_385086141_132000_CN_94816975_132000/RConn1
  T_385086141__/LConn2 -- _CN_385086141_132000_CN_94816975_132000/RConn2
  _CN_385086141_132000_CN_94816975_132000/RConn3 -- T_385086141__/LConn3 -- bus142/LConn1
  T_424681656__/LConn1 -- _CN_424681664_132000_CN_424681656_132000/RConn1
  T_424681656__/LConn2 -- _CN_424681664_132000_CN_424681656_132000/RConn2
  _CN_424681664_132000_CN_424681656_132000/RConn3 -- T_424681656__/LConn3 -- bus143/LConn1
  _CN_424681664_132000_CN_201082863_132000/RConn1 -- T_201082863__/LConn1 -- _CN_188636744_132000_CN_201082863_132000/LConn1
  _CN_424681664_132000_CN_201082863_132000/RConn2 -- T_201082863__/LConn2 -- _CN_188636744_132000_CN_201082863_132000/LConn2
  _CN_424681664_132000_CN_201082863_132000/RConn3 -- T_201082863__/LConn3 -- _CN_188636744_132000_CN_201082863_132000/LConn3 -- bus144/LConn1
  _CN_115677382_132000_CN_115677394_132000/LConn1 -- T_115677382__/LConn1 -- _CN_115677382_132000_CN_115677404_132000/LConn1
  _CN_115677382_132000_CN_115677394_132000/LConn2 -- T_115677382__/LConn2 -- _CN_115677382_132000_CN_115677404_132000/LConn2
  _CN_115677382_132000_CN_115677394_132000/LConn3 -- T_115677382__/LConn3 -- _CN_115677382_132000_CN_115677404_132000/LConn3 -- bus145/LConn1
  _CN_115677382_132000_CN_115677394_132000/RConn1 -- T_115677394__/LConn1 -- _CN_115677383_132000_CN_115677394_132000/LConn1
  _CN_115677382_132000_CN_115677394_132000/RConn2 -- T_115677394__/LConn2 -- _CN_115677383_132000_CN_115677394_132000/LConn2
  _CN_115677382_132000_CN_115677394_132000/RConn3 -- T_115677394__/LConn3 -- _CN_115677383_132000_CN_115677394_132000/LConn3 -- bus146/LConn1
  _CN_115677382_132000_CN_115677404_132000/RConn1 -- T_115677404__/LConn1 -- _CN_115677404_132000_CN_115700870_132000/LConn1
  _CN_115677382_132000_CN_115677404_132000/RConn2 -- T_115677404__/LConn2 -- _CN_115677404_132000_CN_115700870_132000/LConn2
  _CN_115677382_132000_CN_115677404_132000/RConn3 -- T_115677404__/LConn3 -- _CN_115677404_132000_CN_115700870_132000/LConn3 -- bus147/LConn1
  _CN_115677383_132000_CN_115677394_132000/RConn1 -- T_115677383__/RConn1 -- L_115677383/LConn1
  _CN_115677383_132000_CN_115677394_132000/RConn2 -- T_115677383__/RConn2 -- L_115677383/LConn2
  _CN_115677383_132000_CN_115677394_132000/RConn3 -- T_115677383__/RConn3 -- L_115677383/LConn3 -- bus148/LConn1
  T_354672638__/LConn1 -- _CN_354672638_132000_CN_354672635_132000/LConn1
  T_354672638__/LConn2 -- _CN_354672638_132000_CN_354672635_132000/LConn2
  _CN_354672638_132000_CN_354672635_132000/LConn3 -- T_354672638__/LConn3 -- bus149/LConn1
  _CN_354672638_132000_CN_354672635_132000/RConn1 -- T_354672635__/LConn1 -- _CN_386208076_132000_CN_354672635_132000/LConn1
  _CN_354672638_132000_CN_354672635_132000/RConn2 -- T_354672635__/LConn2 -- _CN_386208076_132000_CN_354672635_132000/LConn2
  _CN_354672638_132000_CN_354672635_132000/RConn3 -- T_354672635__/LConn3 -- _CN_386208076_132000_CN_354672635_132000/LConn3 -- bus150/LConn1
  T_203614925__/LConn1 -- _CN_203614925_132000_CN_132889809_132000/LConn1
  T_203614925__/LConn2 -- _CN_203614925_132000_CN_132889809_132000/LConn2
  _CN_203614925_132000_CN_132889809_132000/LConn3 -- T_203614925__/LConn3 -- bus151/LConn1
  _CN_203614925_132000_CN_132889809_132000/RConn1 -- T_132889809__/RConn1 -- _CN_132889809_132000_CN_203979987_132000/LConn1 -- L_132889809/LConn1
  _CN_203614925_132000_CN_132889809_132000/RConn2 -- T_132889809__/RConn2 -- _CN_132889809_132000_CN_203979987_132000/LConn2 -- L_132889809/LConn2
  _CN_203614925_132000_CN_132889809_132000/RConn3 -- T_132889809__/RConn3 -- _CN_132889809_132000_CN_203979987_132000/LConn3 -- L_132889809/LConn3 -- bus152/LConn1
  T_303315256__/LConn1 -- _CN_384752846_132000_CN_303315256_132000/RConn1
  T_303315256__/LConn2 -- _CN_384752846_132000_CN_303315256_132000/RConn2
  _CN_384752846_132000_CN_303315256_132000/RConn3 -- T_303315256__/LConn3 -- bus153/LConn1
  T_303315257__/LConn1 -- _CN_384752846_132000_CN_303315257_132000/RConn1
  T_303315257__/LConn2 -- _CN_384752846_132000_CN_303315257_132000/RConn2
  _CN_384752846_132000_CN_303315257_132000/RConn3 -- T_303315257__/LConn3 -- bus154/LConn1
  G_303315253_/RConn1 -- _CN_384752846_132000_CN_303315253_132000/RConn1
  G_303315253_/RConn2 -- _CN_384752846_132000_CN_303315253_132000/RConn2
  _CN_384752846_132000_CN_303315253_132000/RConn3 -- G_303315253_/RConn3 -- bus155/LConn1
  _CN_115168464_132000_CN_115305410_132000/LConn1 -- T_115168464__/RConn1 -- L_115168464/LConn1
  _CN_115168464_132000_CN_115305410_132000/LConn2 -- T_115168464__/RConn2 -- L_115168464/LConn2
  _CN_115168464_132000_CN_115305410_132000/LConn3 -- T_115168464__/RConn3 -- L_115168464/LConn3 -- bus156/LConn1
  T_115305410__/LConn1 -- _CN_115168464_132000_CN_115305410_132000/RConn1
  T_115305410__/LConn2 -- _CN_115168464_132000_CN_115305410_132000/RConn2
  _CN_115168464_132000_CN_115305410_132000/RConn3 -- T_115305410__/LConn3 -- bus157/LConn1
  T_203979987__/LConn1 -- _CN_132889809_132000_CN_203979987_132000/RConn1
  T_203979987__/LConn2 -- _CN_132889809_132000_CN_203979987_132000/RConn2
  _CN_132889809_132000_CN_203979987_132000/RConn3 -- T_203979987__/LConn3 -- bus158/LConn1
  _CN_115188435_132000_CN_52609391_132000/RConn1 -- T_115188435__/LConn1 -- _CN_115188435_132000_CN_115204753_132000/LConn1
  _CN_115188435_132000_CN_52609391_132000/RConn2 -- T_115188435__/LConn2 -- _CN_115188435_132000_CN_115204753_132000/LConn2
  _CN_115188435_132000_CN_52609391_132000/RConn3 -- T_115188435__/LConn3 -- _CN_115188435_132000_CN_115204753_132000/LConn3 -- bus159/LConn1
  T_115204753__/LConn1 -- _CN_115188435_132000_CN_115204753_132000/RConn1
  T_115204753__/LConn2 -- _CN_115188435_132000_CN_115204753_132000/RConn2
  _CN_115188435_132000_CN_115204753_132000/RConn3 -- T_115204753__/LConn3 -- bus160/LConn1
  T_219620566__substation/LConn1 -- _CN_219620566_132000_CN_295186319_132000/LConn1
  T_219620566__substation/LConn2 -- _CN_219620566_132000_CN_295186319_132000/LConn2
  _CN_219620566_132000_CN_295186319_132000/LConn3 -- T_219620566__substation/LConn3 -- bus161/LConn1
  T_295186319__/LConn1 -- _CN_219620566_132000_CN_295186319_132000/RConn1
  T_295186319__/LConn2 -- _CN_219620566_132000_CN_295186319_132000/RConn2
  _CN_219620566_132000_CN_295186319_132000/RConn3 -- T_295186319__/LConn3 -- bus162/LConn1
  T_181332857__/LConn1 -- _CN_181332857_132000_CN_181332751_132000/LConn1
  T_181332857__/LConn2 -- _CN_181332857_132000_CN_181332751_132000/LConn2
  _CN_181332857_132000_CN_181332751_132000/LConn3 -- T_181332857__/LConn3 -- bus163/LConn1
  _CN_181332857_132000_CN_181332751_132000/RConn1 -- T_181332751__/LConn1 -- _CN_181332751_132000_CN_386063272_132000/LConn1 -- _CN_181332751_132000_CN_181332756_132000/RConn1
  _CN_181332857_132000_CN_181332751_132000/RConn2 -- T_181332751__/LConn2 -- _CN_181332751_132000_CN_386063272_132000/LConn2 -- _CN_181332751_132000_CN_181332756_132000/RConn2
  _CN_181332857_132000_CN_181332751_132000/RConn3 -- T_181332751__/LConn3 -- _CN_181332751_132000_CN_386063272_132000/LConn3 -- _CN_181332751_132000_CN_181332756_132000/RConn3 -- bus164/LConn1
  G_115700870_/RConn1 -- _CN_115677404_132000_CN_115700870_132000/RConn1
  G_115700870_/RConn2 -- _CN_115677404_132000_CN_115700870_132000/RConn2
  _CN_115677404_132000_CN_115700870_132000/RConn3 -- G_115700870_/RConn3 -- bus165/LConn1
  T_204141035__/LConn1 -- _CN_204142303_132000_CN_204141035_132000/RConn1
  T_204141035__/LConn2 -- _CN_204142303_132000_CN_204141035_132000/RConn2
  _CN_204142303_132000_CN_204141035_132000/RConn3 -- T_204141035__/LConn3 -- bus166/LConn1
  _CN_115677414_132000_CN_115677419_132000/LConn1 -- T_115677414__/RConn1 -- _CN_115677414_132000_CN_386138424_132000/LConn1 -- L_115677414/LConn1
  _CN_115677414_132000_CN_115677419_132000/LConn2 -- T_115677414__/RConn2 -- _CN_115677414_132000_CN_386138424_132000/LConn2 -- L_115677414/LConn2
  _CN_115677414_132000_CN_115677419_132000/LConn3 -- T_115677414__/RConn3 -- _CN_115677414_132000_CN_386138424_132000/LConn3 -- L_115677414/LConn3 -- bus167/LConn1
  _CN_115677414_132000_CN_115677419_132000/RConn1 -- T_115677419__/LConn1 -- _CN_115677419_132000_CN_385629058_132000/LConn1
  _CN_115677414_132000_CN_115677419_132000/RConn2 -- T_115677419__/LConn2 -- _CN_115677419_132000_CN_385629058_132000/LConn2
  _CN_115677414_132000_CN_115677419_132000/RConn3 -- T_115677419__/LConn3 -- _CN_115677419_132000_CN_385629058_132000/LConn3 -- bus168/LConn1
  T_386138424__/LConn1 -- _CN_115677414_132000_CN_386138424_132000/RConn1
  T_386138424__/LConn2 -- _CN_115677414_132000_CN_386138424_132000/RConn2
  _CN_115677414_132000_CN_386138424_132000/RConn3 -- T_386138424__/LConn3 -- bus169/LConn1
  G_239581958_/RConn1 -- _CN_239581995_132000_CN_239581958_132000/RConn1
  G_239581958_/RConn2 -- _CN_239581995_132000_CN_239581958_132000/RConn2
  _CN_239581995_132000_CN_239581958_132000/RConn3 -- G_239581958_/RConn3 -- bus170/LConn1
  _CN_115677419_132000_CN_385629058_132000/RConn1 -- T_385629058__/LConn1 -- _CN_39657768_132000_CN_385629058_132000/LConn1
  _CN_115677419_132000_CN_385629058_132000/RConn2 -- T_385629058__/LConn2 -- _CN_39657768_132000_CN_385629058_132000/LConn2
  _CN_115677419_132000_CN_385629058_132000/RConn3 -- T_385629058__/LConn3 -- _CN_39657768_132000_CN_385629058_132000/LConn3 -- bus171/LConn1
  G_239435499_/RConn1 -- _CN_239435500_132000_CN_239435499_132000/RConn1
  G_239435499_/RConn2 -- _CN_239435500_132000_CN_239435499_132000/RConn2
  _CN_239435500_132000_CN_239435499_132000/RConn3 -- G_239435499_/RConn3 -- bus172/LConn1
  T_386202923__/LConn1 -- _CN_386202923_132000_CN_354672632_132000/RConn1
  T_386202923__/LConn2 -- _CN_386202923_132000_CN_354672632_132000/RConn2
  _CN_386202923_132000_CN_354672632_132000/RConn3 -- T_386202923__/LConn3 -- bus173/LConn1
  T_216208125__/LConn1 -- _CN_216208125_132000_CN_115310393_132000/LConn1
  T_216208125__/LConn2 -- _CN_216208125_132000_CN_115310393_132000/LConn2
  _CN_216208125_132000_CN_115310393_132000/LConn3 -- T_216208125__/LConn3 -- bus174/LConn1
  _CN_216208125_132000_CN_115310393_132000/RConn1 -- T_115310393__/LConn1 -- _CN_215091971_132000_CN_115310393_132000/LConn1
  _CN_216208125_132000_CN_115310393_132000/RConn2 -- T_115310393__/LConn2 -- _CN_215091971_132000_CN_115310393_132000/LConn2
  _CN_216208125_132000_CN_115310393_132000/RConn3 -- T_115310393__/LConn3 -- _CN_215091971_132000_CN_115310393_132000/LConn3 -- bus175/LConn1
  T_240323330__/LConn1 -- _CN_240323330_132000_CN_261164502_132000/LConn1
  T_240323330__/LConn2 -- _CN_240323330_132000_CN_261164502_132000/LConn2
  _CN_240323330_132000_CN_261164502_132000/LConn3 -- T_240323330__/LConn3 -- bus176/LConn1
  _CN_240323330_132000_CN_261164502_132000/RConn1 -- T_261164502__/RConn1 -- L_261164502/LConn1
  _CN_240323330_132000_CN_261164502_132000/RConn2 -- T_261164502__/RConn2 -- L_261164502/LConn2
  _CN_240323330_132000_CN_261164502_132000/RConn3 -- T_261164502__/RConn3 -- L_261164502/LConn3 -- bus177/LConn1
  _CN_215091971_132000_CN_208619658_132000/LConn1 -- T_215091971__/LConn1 -- _CN_215091971_132000_CN_115310393_132000/RConn1
  _CN_215091971_132000_CN_208619658_132000/LConn2 -- T_215091971__/LConn2 -- _CN_215091971_132000_CN_115310393_132000/RConn2
  _CN_215091971_132000_CN_208619658_132000/LConn3 -- T_215091971__/LConn3 -- _CN_215091971_132000_CN_115310393_132000/RConn3 -- bus178/LConn1
  _CN_215091971_132000_CN_208619658_132000/RConn1 -- G_208619658_/RConn1 -- _CN_216869978_380000_CN_208619658_132000/LConn1 -- _CN_231599971_380000_CN_208619658_132000/LConn1 -- _CN_215091972_132000_CN_208619658_132000/LConn1 -- _CN_209263045_380000_CN_208619658_132000/LConn1
  _CN_215091971_132000_CN_208619658_132000/RConn2 -- G_208619658_/RConn2 -- _CN_216869978_380000_CN_208619658_132000/LConn2 -- _CN_231599971_380000_CN_208619658_132000/LConn2 -- _CN_215091972_132000_CN_208619658_132000/LConn2 -- _CN_209263045_380000_CN_208619658_132000/LConn2
  _CN_215091971_132000_CN_208619658_132000/RConn3 -- G_208619658_/RConn3 -- _CN_216869978_380000_CN_208619658_132000/LConn3 -- _CN_231599971_380000_CN_208619658_132000/LConn3 -- bus179/LConn1 -- _CN_215091972_132000_CN_208619658_132000/LConn3 -- _CN_209263045_380000_CN_208619658_132000/LConn3
  T_215091972__/LConn1 -- _CN_215091972_132000_CN_208619658_132000/RConn1
  T_215091972__/LConn2 -- _CN_215091972_132000_CN_208619658_132000/RConn2
  _CN_215091972_132000_CN_208619658_132000/RConn3 -- T_215091972__/LConn3 -- bus180/LConn1
  T_386063272__/LConn1 -- _CN_181332751_132000_CN_386063272_132000/RConn1
  T_386063272__/LConn2 -- _CN_181332751_132000_CN_386063272_132000/RConn2
  _CN_181332751_132000_CN_386063272_132000/RConn3 -- T_386063272__/LConn3 -- bus181/LConn1
  _CN_260963603_132000_CN_240292205_132000/LConn1 -- T_260963603__/RConn1 -- _CN_260963603_132000_CN_181332756_132000/RConn1 -- _CN_260963603_132000_CN_385263258_132000/RConn1 -- L_260963603/LConn1 -- _CN_260963603_132000_CN_220817213_132000/RConn1 -- _CN_260963603_132000_CN_240292204_132000/LConn1
  _CN_260963603_132000_CN_240292205_132000/LConn2 -- T_260963603__/RConn2 -- _CN_260963603_132000_CN_181332756_132000/RConn2 -- _CN_260963603_132000_CN_385263258_132000/RConn2 -- L_260963603/LConn2 -- _CN_260963603_132000_CN_220817213_132000/RConn2 -- _CN_260963603_132000_CN_240292204_132000/LConn2
  _CN_260963603_132000_CN_240292205_132000/LConn3 -- T_260963603__/RConn3 -- _CN_260963603_132000_CN_181332756_132000/RConn3 -- _CN_260963603_132000_CN_385263258_132000/RConn3 -- L_260963603/LConn3 -- bus182/LConn1 -- _CN_260963603_132000_CN_220817213_132000/RConn3 -- _CN_260963603_132000_CN_240292204_132000/LConn3
  T_240292205__/LConn1 -- _CN_260963603_132000_CN_240292205_132000/RConn1
  T_240292205__/LConn2 -- _CN_260963603_132000_CN_240292205_132000/RConn2
  _CN_260963603_132000_CN_240292205_132000/RConn3 -- T_240292205__/LConn3 -- bus183/LConn1
  T_240292204__/LConn1 -- _CN_260963603_132000_CN_240292204_132000/RConn1
  T_240292204__/LConn2 -- _CN_260963603_132000_CN_240292204_132000/RConn2
  _CN_260963603_132000_CN_240292204_132000/RConn3 -- T_240292204__/LConn3 -- bus184/LConn1
  T_239679334__/LConn1 -- _CN_239679266_132000_CN_239679334_132000/RConn1
  T_239679334__/LConn2 -- _CN_239679266_132000_CN_239679334_132000/RConn2
  _CN_239679266_132000_CN_239679334_132000/RConn3 -- T_239679334__/LConn3 -- bus185/LConn1
  _CN_39657768_132000_CN_385629058_132000/RConn1 -- T_39657768__/LConn1 -- _CN_39657768_132000_CN_115677372_132000/RConn1
  _CN_39657768_132000_CN_385629058_132000/RConn2 -- T_39657768__/LConn2 -- _CN_39657768_132000_CN_115677372_132000/RConn2
  _CN_39657768_132000_CN_385629058_132000/RConn3 -- T_39657768__/LConn3 -- _CN_39657768_132000_CN_115677372_132000/RConn3 -- bus186/LConn1
  T_115797300__/LConn1 -- _CN_115797297_132000_CN_115797300_132000/RConn1
  T_115797300__/LConn2 -- _CN_115797297_132000_CN_115797300_132000/RConn2
  _CN_115797297_132000_CN_115797300_132000/RConn3 -- T_115797300__/LConn3 -- bus187/LConn1
  T_385499970__/LConn1 -- _CN_385499970_132000_CN_203975634_132000/LConn1
  T_385499970__/LConn2 -- _CN_385499970_132000_CN_203975634_132000/LConn2
  _CN_385499970_132000_CN_203975634_132000/LConn3 -- T_385499970__/LConn3 -- bus188/LConn1
  T_203975634__/LConn1 -- _CN_385499970_132000_CN_203975634_132000/RConn1
  T_203975634__/LConn2 -- _CN_385499970_132000_CN_203975634_132000/RConn2
  _CN_385499970_132000_CN_203975634_132000/RConn3 -- T_203975634__/LConn3 -- bus189/LConn1
  T_369326404__/LConn1 -- _CN_369326404_132000_CN_190221972_132000/LConn1
  T_369326404__/LConn2 -- _CN_369326404_132000_CN_190221972_132000/LConn2
  _CN_369326404_132000_CN_190221972_132000/LConn3 -- T_369326404__/LConn3 -- bus190/LConn1
  _CN_369326404_132000_CN_190221972_132000/RConn1 -- T_190221972__/LConn1 -- _CN_190221972_132000_CN_167842250_132000/LConn1 -- _CN_190221972_132000_CN_188636744_132000/LConn1
  _CN_369326404_132000_CN_190221972_132000/RConn2 -- T_190221972__/LConn2 -- _CN_190221972_132000_CN_167842250_132000/LConn2 -- _CN_190221972_132000_CN_188636744_132000/LConn2
  _CN_369326404_132000_CN_190221972_132000/RConn3 -- T_190221972__/LConn3 -- _CN_190221972_132000_CN_167842250_132000/LConn3 -- _CN_190221972_132000_CN_188636744_132000/LConn3 -- bus191/LConn1
  T_240577351__/LConn1 -- _CN_240577351_132000_CN_384716522_132000/LConn1
  T_240577351__/LConn2 -- _CN_240577351_132000_CN_384716522_132000/LConn2
  _CN_240577351_132000_CN_384716522_132000/LConn3 -- T_240577351__/LConn3 -- bus192/LConn1
  T_384716522__/LConn1 -- _CN_240577351_132000_CN_384716522_132000/RConn1
  T_384716522__/LConn2 -- _CN_240577351_132000_CN_384716522_132000/RConn2
  _CN_240577351_132000_CN_384716522_132000/RConn3 -- T_384716522__/LConn3 -- bus193/LConn1
  T_168661559__/LConn1 -- _CN_168661559_132000_CN_188636744_132000/LConn1
  T_168661559__/LConn2 -- _CN_168661559_132000_CN_188636744_132000/LConn2
  _CN_168661559_132000_CN_188636744_132000/LConn3 -- T_168661559__/LConn3 -- bus194/LConn1
  _CN_168661559_132000_CN_188636744_132000/RConn1 -- T_188636744__/LConn1 -- _CN_190221972_132000_CN_188636744_132000/RConn1 -- _CN_188636744_132000_CN_201082863_132000/RConn1
  _CN_168661559_132000_CN_188636744_132000/RConn2 -- T_188636744__/LConn2 -- _CN_190221972_132000_CN_188636744_132000/RConn2 -- _CN_188636744_132000_CN_201082863_132000/RConn2
  _CN_168661559_132000_CN_188636744_132000/RConn3 -- T_188636744__/LConn3 -- _CN_190221972_132000_CN_188636744_132000/RConn3 -- _CN_188636744_132000_CN_201082863_132000/RConn3 -- bus195/LConn1
  T_386208076__/LConn1 -- _CN_386208076_132000_CN_354672635_132000/RConn1
  T_386208076__/LConn2 -- _CN_386208076_132000_CN_354672635_132000/RConn2
  _CN_386208076_132000_CN_354672635_132000/RConn3 -- T_386208076__/LConn3 -- bus196/LConn1
  _CN_121847629_132000_CN_181133259_132000/RConn1 -- T_181133259__/LConn1 -- _CN_181133259_132000_CN_199713782_132000/LConn1
  _CN_121847629_132000_CN_181133259_132000/RConn2 -- T_181133259__/LConn2 -- _CN_181133259_132000_CN_199713782_132000/LConn2
  _CN_121847629_132000_CN_181133259_132000/RConn3 -- T_181133259__/LConn3 -- _CN_181133259_132000_CN_199713782_132000/LConn3 -- bus197/LConn1
  T_167842250__/LConn1 -- _CN_190221972_132000_CN_167842250_132000/RConn1
  T_167842250__/LConn2 -- _CN_190221972_132000_CN_167842250_132000/RConn2
  _CN_190221972_132000_CN_167842250_132000/RConn3 -- T_167842250__/LConn3 -- bus198/LConn1
  T_384688538__/LConn1 -- _CN_384688538_132000_CN_239990697_132000/RConn1
  T_384688538__/LConn2 -- _CN_384688538_132000_CN_239990697_132000/RConn2
  _CN_384688538_132000_CN_239990697_132000/RConn3 -- T_384688538__/LConn3 -- bus199/LConn1
  T_181132699__/LConn1 -- _CN_181132699_132000_CN_181132741_132000/RConn1
  T_181132699__/LConn2 -- _CN_181132699_132000_CN_181132741_132000/RConn2
  _CN_181132699_132000_CN_181132741_132000/RConn3 -- T_181132699__/LConn3 -- bus200/LConn1
  T_384688544__/LConn1 -- _CN_239990697_132000_CN_384688544_132000/RConn1
  T_384688544__/LConn2 -- _CN_239990697_132000_CN_384688544_132000/RConn2
  _CN_239990697_132000_CN_384688544_132000/RConn3 -- T_384688544__/LConn3 -- bus201/LConn1
  T_384731081__/LConn1 -- _CN_384731081_132000_CN_240045481_132000/RConn1
  T_384731081__/LConn2 -- _CN_384731081_132000_CN_240045481_132000/RConn2
  _CN_384731081_132000_CN_240045481_132000/RConn3 -- T_384731081__/LConn3 -- bus202/LConn1
  T_199713782__/LConn1 -- _CN_181133259_132000_CN_199713782_132000/RConn1
  T_199713782__/LConn2 -- _CN_181133259_132000_CN_199713782_132000/RConn2
  _CN_181133259_132000_CN_199713782_132000/RConn3 -- T_199713782__/LConn3 -- bus203/LConn1
  _CN_29504133_220000_CN_94950857_220000/LConn1 -- T_29504133__Substation/LConn1 -- _CN_29504133_220000_CN_95046964_220000/LConn1 -- _CN_29504133_220000_CN_95046332_220000/LConn1 -- _CN_29504133_220000_CN_29504119_220000/LConn1 -- _CN_29504133_220000_CN_29503687_220000/LConn1 -- _CN_29504133_220000_CN_24394891_220000/LConn1
  _CN_29504133_220000_CN_94950857_220000/LConn2 -- T_29504133__Substation/LConn2 -- _CN_29504133_220000_CN_95046964_220000/LConn2 -- _CN_29504133_220000_CN_95046332_220000/LConn2 -- _CN_29504133_220000_CN_29504119_220000/LConn2 -- _CN_29504133_220000_CN_29503687_220000/LConn2 -- _CN_29504133_220000_CN_24394891_220000/LConn2
  _CN_29504133_220000_CN_94950857_220000/LConn3 -- T_29504133__Substation/LConn3 -- _CN_29504133_220000_CN_95046964_220000/LConn3 -- bus204/LConn1 -- _CN_29504133_220000_CN_95046332_220000/LConn3 -- _CN_29504133_220000_CN_29504119_220000/LConn3 -- _CN_29504133_220000_CN_29503687_220000/LConn3 -- _CN_29504133_220000_CN_24394891_220000/LConn3
  T_94950857__/LConn1 -- _CN_29504133_220000_CN_94950857_220000/RConn1
  T_94950857__/LConn2 -- _CN_29504133_220000_CN_94950857_220000/RConn2
  _CN_29504133_220000_CN_94950857_220000/RConn3 -- T_94950857__/LConn3 -- bus205/LConn1
  _CN_29504133_220000_CN_95046332_220000/RConn1 -- T_95046332__Mussafah_GIC_Substation/LConn1 -- _CN_95046332_220000_CN_259874704_220000/LConn1 -- _CN_95046332_220000_CN_29504119_220000/LConn1
  _CN_29504133_220000_CN_95046332_220000/RConn2 -- T_95046332__Mussafah_GIC_Substation/LConn2 -- _CN_95046332_220000_CN_259874704_220000/LConn2 -- _CN_95046332_220000_CN_29504119_220000/LConn2
  _CN_29504133_220000_CN_95046332_220000/RConn3 -- T_95046332__Mussafah_GIC_Substation/LConn3 -- _CN_95046332_220000_CN_259874704_220000/LConn3 -- _CN_95046332_220000_CN_29504119_220000/LConn3 -- bus206/LConn1
  _CN_29504133_220000_CN_29504119_220000/RConn1 -- T_29504119__Substation/RConn1 -- _CN_95046332_220000_CN_29504119_220000/RConn1 -- L_29504119/LConn1
  _CN_29504133_220000_CN_29504119_220000/RConn2 -- T_29504119__Substation/RConn2 -- _CN_95046332_220000_CN_29504119_220000/RConn2 -- L_29504119/LConn2
  _CN_29504133_220000_CN_29504119_220000/RConn3 -- T_29504119__Substation/RConn3 -- _CN_95046332_220000_CN_29504119_220000/RConn3 -- L_29504119/LConn3 -- bus207/LConn1
  T_29503687__Substation/LConn1 -- _CN_29504133_220000_CN_29503687_220000/RConn1
  T_29503687__Substation/LConn2 -- _CN_29504133_220000_CN_29503687_220000/RConn2
  _CN_29504133_220000_CN_29503687_220000/RConn3 -- T_29503687__Substation/LConn3 -- bus208/LConn1
  _CN_29504133_220000_CN_24394891_220000/RConn1 -- T_24394891__/RConn1 -- L_24394891/LConn1
  _CN_29504133_220000_CN_24394891_220000/RConn2 -- T_24394891__/RConn2 -- L_24394891/LConn2
  _CN_29504133_220000_CN_24394891_220000/RConn3 -- T_24394891__/RConn3 -- L_24394891/LConn3 -- bus209/LConn1
  _CN_29504133_220000_CN_95046964_220000/RConn1 -- T_95046964__Khazna/LConn1 -- _CN_95055625_220000_CN_95046964_220000/LConn1
  _CN_29504133_220000_CN_95046964_220000/RConn2 -- T_95046964__Khazna/LConn2 -- _CN_95055625_220000_CN_95046964_220000/LConn2
  _CN_29504133_220000_CN_95046964_220000/RConn3 -- T_95046964__Khazna/LConn3 -- _CN_95055625_220000_CN_95046964_220000/LConn3 -- bus210/LConn1
  T_261164502__/LConn1 -- _CN_261164502_220000_CN_95084794_220000/LConn1
  T_261164502__/LConn2 -- _CN_261164502_220000_CN_95084794_220000/LConn2
  _CN_261164502_220000_CN_95084794_220000/LConn3 -- T_261164502__/LConn3 -- bus211/LConn1
  _CN_261164502_220000_CN_95084794_220000/RConn1 -- T_95084794__/LConn1 -- _CN_95084794_220000_CN_95084799_220000/LConn1
  _CN_261164502_220000_CN_95084794_220000/RConn2 -- T_95084794__/LConn2 -- _CN_95084794_220000_CN_95084799_220000/LConn2
  _CN_261164502_220000_CN_95084794_220000/RConn3 -- T_95084794__/LConn3 -- _CN_95084794_220000_CN_95084799_220000/LConn3 -- bus212/LConn1
  _CN_95055625_220000_CN_95046964_220000/RConn1 -- T_95055625__Ramah/LConn1 -- _CN_95055625_220000_CN_95084816_220000/LConn1
  _CN_95055625_220000_CN_95046964_220000/RConn2 -- T_95055625__Ramah/LConn2 -- _CN_95055625_220000_CN_95084816_220000/LConn2
  _CN_95055625_220000_CN_95046964_220000/RConn3 -- T_95055625__Ramah/LConn3 -- _CN_95055625_220000_CN_95084816_220000/LConn3 -- bus213/LConn1
  _CN_95055625_220000_CN_95084816_220000/RConn1 -- T_95084816__/LConn1 -- _CN_95084816_220000_CN_200057688_220000/LConn1 -- _CN_95084816_220000_CN_95097245_220000/LConn1 -- _CN_95084816_220000_CN_95084811_220000/LConn1 -- _CN_95084816_220000_CN_132159924_220000/LConn1
  _CN_95055625_220000_CN_95084816_220000/RConn2 -- T_95084816__/LConn2 -- _CN_95084816_220000_CN_200057688_220000/LConn2 -- _CN_95084816_220000_CN_95097245_220000/LConn2 -- _CN_95084816_220000_CN_95084811_220000/LConn2 -- _CN_95084816_220000_CN_132159924_220000/LConn2
  _CN_95055625_220000_CN_95084816_220000/RConn3 -- T_95084816__/LConn3 -- _CN_95084816_220000_CN_200057688_220000/LConn3 -- _CN_95084816_220000_CN_95097245_220000/LConn3 -- _CN_95084816_220000_CN_95084811_220000/LConn3 -- _CN_95084816_220000_CN_132159924_220000/LConn3 -- bus214/LConn1
  _CN_95084816_220000_CN_200057688_220000/RConn1 -- T_200057688__AASW/LConn1 -- _CN_181362976_220000_CN_200057688_220000/LConn1 -- _CN_95084811_220000_CN_200057688_220000/LConn1 -- _CN_200057688_220000_CN_95084793_220000/LConn1
  _CN_95084816_220000_CN_200057688_220000/RConn2 -- T_200057688__AASW/LConn2 -- _CN_181362976_220000_CN_200057688_220000/LConn2 -- _CN_95084811_220000_CN_200057688_220000/LConn2 -- _CN_200057688_220000_CN_95084793_220000/LConn2
  _CN_95084816_220000_CN_200057688_220000/RConn3 -- T_200057688__AASW/LConn3 -- _CN_181362976_220000_CN_200057688_220000/LConn3 -- _CN_95084811_220000_CN_200057688_220000/LConn3 -- _CN_200057688_220000_CN_95084793_220000/LConn3 -- bus215/LConn1
  T_95097245__Al_Wagon/LConn1 -- _CN_95084816_220000_CN_95097245_220000/RConn1
  T_95097245__Al_Wagon/LConn2 -- _CN_95084816_220000_CN_95097245_220000/RConn2
  _CN_95084816_220000_CN_95097245_220000/RConn3 -- T_95097245__Al_Wagon/LConn3 -- bus216/LConn1
  _CN_95084816_220000_CN_95084811_220000/RConn1 -- T_95084811__Arad/LConn1 -- _CN_95084811_220000_CN_200057688_220000/RConn1
  _CN_95084816_220000_CN_95084811_220000/RConn2 -- T_95084811__Arad/LConn2 -- _CN_95084811_220000_CN_200057688_220000/RConn2
  _CN_95084816_220000_CN_95084811_220000/RConn3 -- T_95084811__Arad/LConn3 -- _CN_95084811_220000_CN_200057688_220000/RConn3 -- bus217/LConn1
  T_132159924__Umm_Al_Oush/LConn1 -- _CN_95084816_220000_CN_132159924_220000/RConn1
  T_132159924__Umm_Al_Oush/LConn2 -- _CN_95084816_220000_CN_132159924_220000/RConn2
  _CN_95084816_220000_CN_132159924_220000/RConn3 -- T_132159924__Umm_Al_Oush/LConn3 -- bus218/LConn1
  T_29500305__/LConn1 -- _CN_29500305_220000_CN_29499064_220000/LConn1
  T_29500305__/LConn2 -- _CN_29500305_220000_CN_29499064_220000/LConn2
  _CN_29500305_220000_CN_29499064_220000/LConn3 -- T_29500305__/LConn3 -- bus219/LConn1
  _CN_29500305_220000_CN_29499064_220000/RConn1 -- T_29499064__/LConn1 -- _CN_181332756_220000_CN_29499064_220000/LConn1
  _CN_29500305_220000_CN_29499064_220000/RConn2 -- T_29499064__/LConn2 -- _CN_181332756_220000_CN_29499064_220000/LConn2
  _CN_29500305_220000_CN_29499064_220000/RConn3 -- T_29499064__/LConn3 -- _CN_181332756_220000_CN_29499064_220000/LConn3 -- bus220/LConn1
  T_181332756__/RConn1 -- _CN_181332756_220000_CN_29499064_220000/RConn1
  T_181332756__/RConn2 -- _CN_181332756_220000_CN_29499064_220000/RConn2
  _CN_181332756_220000_CN_29499064_220000/RConn3 -- T_181332756__/RConn3 -- bus221/LConn1
  _CN_181362976_220000_CN_95084771_220000/LConn1 -- T_181362976__Substation/LConn1 -- _CN_181362976_220000_CN_200057688_220000/RConn1
  _CN_181362976_220000_CN_95084771_220000/LConn2 -- T_181362976__Substation/LConn2 -- _CN_181362976_220000_CN_200057688_220000/RConn2
  _CN_181362976_220000_CN_95084771_220000/LConn3 -- T_181362976__Substation/LConn3 -- _CN_181362976_220000_CN_200057688_220000/RConn3 -- bus222/LConn1
  _CN_181362976_220000_CN_95084771_220000/RConn1 -- T_95084771__/LConn1 -- _CN_95084771_220000_CN_95084793_220000/LConn1
  _CN_181362976_220000_CN_95084771_220000/RConn2 -- T_95084771__/LConn2 -- _CN_95084771_220000_CN_95084793_220000/LConn2
  _CN_181362976_220000_CN_95084771_220000/RConn3 -- T_95084771__/LConn3 -- _CN_95084771_220000_CN_95084793_220000/LConn3 -- bus223/LConn1
  T_95097252__Dabiya/LConn1 -- _CN_95097252_220000_CN_181332765_220000/LConn1
  T_95097252__Dabiya/LConn2 -- _CN_95097252_220000_CN_181332765_220000/LConn2
  _CN_95097252_220000_CN_181332765_220000/LConn3 -- T_95097252__Dabiya/LConn3 -- bus224/LConn1
  _CN_95097252_220000_CN_181332765_220000/RConn1 -- T_181332765__Central/LConn1 -- _CN_181332765_220000_CN_259874704_220000/LConn1 -- _CN_215795245_220000_CN_181332765_220000/LConn1
  _CN_95097252_220000_CN_181332765_220000/RConn2 -- T_181332765__Central/LConn2 -- _CN_181332765_220000_CN_259874704_220000/LConn2 -- _CN_215795245_220000_CN_181332765_220000/LConn2
  _CN_95097252_220000_CN_181332765_220000/RConn3 -- T_181332765__Central/LConn3 -- _CN_181332765_220000_CN_259874704_220000/LConn3 -- bus225/LConn1 -- _CN_215795245_220000_CN_181332765_220000/LConn3
  _CN_95046953_220000_CN_95084799_220000/LConn1 -- T_95046953__Sweihan/RConn1 -- _CN_95046953_220000_CN_95084776_220000/LConn1 -- L_95046953/LConn1
  _CN_95046953_220000_CN_95084799_220000/LConn2 -- T_95046953__Sweihan/RConn2 -- _CN_95046953_220000_CN_95084776_220000/LConn2 -- L_95046953/LConn2
  _CN_95046953_220000_CN_95084799_220000/LConn3 -- T_95046953__Sweihan/RConn3 -- _CN_95046953_220000_CN_95084776_220000/LConn3 -- L_95046953/LConn3 -- bus226/LConn1
  _CN_95046953_220000_CN_95084799_220000/RConn1 -- T_95084799__Dahma/RConn1 -- _CN_95084794_220000_CN_95084799_220000/RConn1 -- L_95084799/LConn1
  _CN_95046953_220000_CN_95084799_220000/RConn2 -- T_95084799__Dahma/RConn2 -- _CN_95084794_220000_CN_95084799_220000/RConn2 -- L_95084799/LConn2
  _CN_95046953_220000_CN_95084799_220000/RConn3 -- T_95084799__Dahma/RConn3 -- _CN_95084794_220000_CN_95084799_220000/RConn3 -- L_95084799/LConn3 -- bus227/LConn1
  T_95084776__/LConn1 -- _CN_95046953_220000_CN_95084776_220000/RConn1
  T_95084776__/LConn2 -- _CN_95046953_220000_CN_95084776_220000/RConn2
  _CN_95046953_220000_CN_95084776_220000/RConn3 -- T_95084776__/LConn3 -- bus228/LConn1
  T_115677383__/LConn1 -- _CN_115677383_220000_CN_354672631_220000/LConn1
  T_115677383__/LConn2 -- _CN_115677383_220000_CN_354672631_220000/LConn2
  _CN_115677383_220000_CN_354672631_220000/LConn3 -- T_115677383__/LConn3 -- bus229/LConn1
  _CN_115677383_220000_CN_354672631_220000/RConn1 -- T_354672631__/LConn1 -- _CN_354672631_220000_CN_115677414_220000/LConn1
  _CN_115677383_220000_CN_354672631_220000/RConn2 -- T_354672631__/LConn2 -- _CN_354672631_220000_CN_115677414_220000/LConn2
  _CN_115677383_220000_CN_354672631_220000/RConn3 -- T_354672631__/LConn3 -- _CN_354672631_220000_CN_115677414_220000/LConn3 -- bus230/LConn1
  T_215795245__Rumaithy/LConn1 -- _CN_215795245_220000_CN_181332765_220000/RConn1
  T_215795245__Rumaithy/LConn2 -- _CN_215795245_220000_CN_181332765_220000/RConn2
  _CN_215795245_220000_CN_181332765_220000/RConn3 -- T_215795245__Rumaithy/LConn3 -- bus231/LConn1
  _CN_181332765_220000_CN_259874704_220000/RConn1 -- T_259874704__/RConn1 -- _CN_95046332_220000_CN_259874704_220000/RConn1 -- L_259874704/LConn1
  _CN_181332765_220000_CN_259874704_220000/RConn2 -- T_259874704__/RConn2 -- _CN_95046332_220000_CN_259874704_220000/RConn2 -- L_259874704/LConn2
  _CN_181332765_220000_CN_259874704_220000/RConn3 -- T_259874704__/RConn3 -- _CN_95046332_220000_CN_259874704_220000/RConn3 -- L_259874704/LConn3 -- bus232/LConn1
  T_181361589__Asab/LConn1 -- _CN_181361589_220000_CN_95099964_220000/LConn1
  T_181361589__Asab/LConn2 -- _CN_181361589_220000_CN_95099964_220000/LConn2
  _CN_181361589_220000_CN_95099964_220000/LConn3 -- T_181361589__Asab/LConn3 -- bus233/LConn1
  _CN_181361589_220000_CN_95099964_220000/RConn1 -- T_95099964__Madinat_Zayed/LConn1 -- _CN_95099973_220000_CN_95099964_220000/LConn1 -- _CN_95099964_220000_CN_95139199_220000/LConn1
  _CN_181361589_220000_CN_95099964_220000/RConn2 -- T_95099964__Madinat_Zayed/LConn2 -- _CN_95099973_220000_CN_95099964_220000/LConn2 -- _CN_95099964_220000_CN_95139199_220000/LConn2
  _CN_181361589_220000_CN_95099964_220000/RConn3 -- T_95099964__Madinat_Zayed/LConn3 -- _CN_95099973_220000_CN_95099964_220000/LConn3 -- _CN_95099964_220000_CN_95139199_220000/LConn3 -- bus234/LConn1
  T_132159930__Sila/LConn1 -- _CN_132159930_220000_CN_132517028_220000/LConn1
  T_132159930__Sila/LConn2 -- _CN_132159930_220000_CN_132517028_220000/LConn2
  _CN_132159930_220000_CN_132517028_220000/LConn3 -- T_132159930__Sila/LConn3 -- bus235/LConn1
  _CN_132159930_220000_CN_132517028_220000/RConn1 -- T_132517028__Ruwais/LConn1 -- _CN_95139157_220000_CN_132517028_220000/LConn1
  _CN_132159930_220000_CN_132517028_220000/RConn2 -- T_132517028__Ruwais/LConn2 -- _CN_95139157_220000_CN_132517028_220000/LConn2
